simulink model "Control_test"  (R2014b)
settings: Solver=FixedStepDiscrete  StartTime=0.0  StopTime=Inf  FixedStep=0.001  RelTol=1e-3
PostLoadFcn:
  | , if any(exist('dsrtsu_mdlpostloadfcn', 'file') == [2, 3, 6]), try dsrtsu_mdlpostloadfcn('Execute', bdroot); catch fprintf('Error in PostLoadFcn (dsrtsu_mdlpostloadfcn) for model "%s":\n %s\n', bdroot, lasterr); end, end,
undefined symbols (not defined in the file or in its folder): dtLocal, slcm
libraries: rtican x163, simulink x14
(part 16 of 34)

== system Control_test/InputProcessing/RadarCanProcessing/MotionPower ==
  Bus Creator : BusCreator  Inputs=258
  Bus Creator1 : BusCreator  Inputs=64
  Bus Selector : BusSelector  OutputSignals=CAN_TX_TRACK_MOVING01,CAN_TX_TRACK_MOVING02,CAN_TX_TRACK_MOVING03,CAN_TX_TRACK_MOVING04,CAN_TX_TRACK_MOVING05,CAN_TX_TRACK_MOVING06,CAN_TX_TRACK_MOVING07,CAN_TX_TRACK_MOVING08,CAN_TX_TRACK_MOVING09,CAN_TX_TRACK_MOVING10,CAN_TX_TRACK_MOVING11,CAN_TX_TRACK_MOVING12,CAN_TX_TRACK_MOVING13,CAN_TX_TRACK_MOVING14,CAN_TX_TRACK_MOVING15,CAN_TX_TRACK_MOVING16,CAN_TX_TRACK_MOVING17,CAN_TX_TRACK_MOVING18,CAN_TX_TRACK_MOVING19,CAN_TX_TRACK_MOVING20,CAN_TX_TRACK_MOVING21,CAN_TX_TRACK_MOVING22,CAN_TX_TRACK_MOVING23,CAN_TX_TRACK_MOVING24,CAN_TX_TRACK_MOVING25,CAN_TX_TRACK_MOVING26,CAN_TX_TRACK_MOVING27,CAN_TX_TRACK_MOVING28,CAN_TX_TRACK_MOVING29,CAN_TX_TRACK_MOVING30,CAN_TX_TRACK_MOVING31,CAN_TX_TRACK_MOVING32,CAN_TX_TRACK_MOVING33,CAN_TX_TRACK_MOVING34,CAN_TX_TRACK_MOVING35,CAN_TX_TRACK_MOVING36,CAN_TX_TRACK_MOVING37,CAN_TX_TRACK_MOVING38,CAN_TX_TRACK_MOVING39,CAN_TX_TRACK_MOVING40,CAN_TX_TRACK_MOVING41,CAN_TX_TRACK_MOVING42,CAN_TX_TRACK_MOVING43,CAN_TX_TRACK_MOVING44,CAN_TX_TRACK_MOVING45,CAN_TX_TRACK_MOVING46,CAN_TX_TRACK_MOVING47,CAN_TX_TRACK_MOVING48,CAN_TX_TRACK_MOVING49,CAN_TX_TRACK_MOVING50,CAN_TX_TRACK_MOVING51,CAN_TX_TRACK_MOVING52,CAN_TX_TRACK_MOVING53,CAN_TX_TRACK_MOVING54,CAN_TX_TRACK_MOVING55,CAN_TX_TRACK_MOVING56,CAN_TX_TRACK_MOVING57,CAN_TX_TRACK_MOVING58,CAN_TX_TRACK_MOVING59,CAN_TX_TRACK_MOVING60,CAN_TX_TRACK_MOVING61,CAN_TX_TRACK_MOVING62,CAN_TX_TRACK_MOVING63,CAN_TX_TRACK_MOVING64
  ESR_TrackMotionPower : rtican/RTICAN Receive (RX)   Reserved1=[]  Reserved2=[]  Reserved3=[]  Reserved4=[]  SfcnMessage=[]  Msg_Struct=[]  BoardTypeNo=[]  BoardNo=[]  ChannelNo=[]  Parameters=[]  DialogFcn=[]  UnitName=[]  Revision=[]  UnitValues=[]  DSProperties=struct('RTI',struct('Version',uint32(5),'BlockType',struct('isSLSource',uint8(1),'isSLSink',uint8(1),'isHWSource',uint8(0),'isHWSink',uint8(0),'isSetup',uint8(0),'isInline',uint8(1),'isNonInline',uint8(0),'isInterrupt',uint8(0),'isChannelwise',uint8(0)),'IOBoardType','RTICAN','UnitType','MESSAGE','Identifier','RX','DialogType','MSVC','BlockSet','RTICAN','SlaveProcessor','CAN'))  RTIBlockInterface=struct('OutputPortsWidth',int32([1 1 1 1 1 1 1 1 1 1 1 1 1 1 1 1 1 1 1 1 1 1 1 1 1 1 1 1 1 1 1 1 1 1 1 1 1 1 1 1 1 1 1 1 1 1 1 1 1 1 1 1 1 1 1 1 1 1 1 1 1 1 1 1 1 1 1 1 1 1 1 1 1 1 1 1 1 1 1 1 1 1 1 1 1 1 1 1 1 1 1 1 1 1 1 1 1 1 1 1 1 1 1 1 1 1 1 1 1 1 1 1 1 1 1 1 1 1 1 1 1 1 1 1 1 1 1 1 1 1 1 1 1 1 1 1 1 1 1 1 1 1 1 1 1 1 1 1 1 1 1 1 1 1 1 1 1 1 1 1 1 1 1 1 1 1 1 1 1 1 1 1 1 1 1 1 1 1 1 1 1 1 1 1 1 1 1 1 1 1 1 1 1 1 1 1 1 1 1 1 1 1 1 1 1 1 1 1 1 1 1 1 1 1 1 1 1 1 1 1 1 1 1 1 1 1 1 1 1 1 1 1 1 1 1 1 1 1 1 1 1 1 1 1 1 1 1 1 1 1 1 1 1 1 1 1 1 1]),'OutputPortsActive',[1 1 1 1 1 1 1 1 1 1 1 1 1 1 1 1 1 1 1 1 1 1 1 1 1 1 1 1 1 1 1 1 1 1 1 1 1 1 1 1 1 1 1 1 1 1 1 1 1 1 1 1 1 1 1 1 1 1 1 1 1 1 1 1 1 1 1 1 1 1 1 1 1 1 1 1 1 1 1 1 1 1 1 1 1 1 1 1 1 1 1 1 1 1 1 1 1 1 1 1 1 1 1 1 1 1 1 1 1 1 1 1 1 1 1 1 1 1 1 1 1 1 1 1 1 1 1 1 1 1 1 1 1 1 1 1 1 1 1 1 1 1 1 1 1 1 1 1 1 1 1 1 1 1 1 1 1 1 1 1 1 1 1 1 1 1 1 1 1 1 1 1 1 1 1 1 1 1 1 1 1 1 1 1 1 1 1 1 1 1 1 1 1 1 1 1 1 1 1 1 1 1 1 1 1 1 1 1 1 1 1 1 1 1 1 1 1 1 1 1 1 1 1 1 1 1 1 1 1 1 1 1 1 1 1 1 1 1 1 1 1 1 1 1 1 1 1 1 1 1 1 1 1 1 1 1 1 1],'OutputPortsName',{{'CAN_TX_TRACK_POWER07','CAN_TX_TRACK_POWER14','CAN_TX_TRACK_POWER21','CAN_TX_TRACK_POWER28','CAN_TX_TRACK_POWER35','CAN_TX_TRACK_POWER42','CAN_TX_TRACK_POWER49','CAN_TX_TRACK_POWER56','CAN_TX_TRACK_POWER63','CAN_TX_TRACK_MOVING07','CAN_TX_TRACK_MOVING14','CAN_TX_TRACK_MOVING21','CAN_TX_TRACK_MOVING28','CAN_TX_TRACK_MOVING35','CAN_TX_TRACK_MOVING42','CAN_TX_TRACK_MOVING49','CAN_TX_TRACK_MOVING56','CAN_TX_TRACK_MOVING63','CAN_TX_TRACK_MOVABLE_SLOW07','CAN_TX_TRACK_MOVABLE_SLOW14','CAN_TX_TRACK_MOVABLE_SLOW21','CAN_TX_TRACK_MOVABLE_SLOW28','CAN_TX_TRACK_MOVABLE_SLOW35','CAN_TX_TRACK_MOVABLE_SLOW42','CAN_TX_TRACK_MOVABLE_SLOW49','CAN_TX_TRACK_MOVABLE_SLOW56','CAN_TX_TRACK_MOVABLE_SLOW63','CAN_TX_TRACK_MOVABLE_FAST07','CAN_TX_TRACK_MOVABLE_FAST14','CAN_TX_TRACK_MOVABLE_FAST21','CAN_TX_TRACK_MOVABLE_FAST28','CAN_TX_TRACK_MOVABLE_FAST35','CAN_TX_TRACK_MOVABLE_FAST42','CAN_TX_TRACK_MOVABLE_FAST49','CAN_TX_TRACK_MOVABLE_FAST56','CAN_TX_TRACK_MOVABLE_FAST63','CAN_TX_TRACK_POWER06','CAN_TX_TRACK_POWER13','CAN_TX_TRACK_POWER20','CAN_TX_TRACK_POWER27','CAN_TX_TRACK_POWER34','CAN_TX_TRACK_POWER41','CAN_TX_TRACK_POWER48','CAN_TX_TRACK_POWER55','CAN_TX_TRACK_POWER62','CAN_TX_TRACK_MOVING06','CAN_TX_TRACK_MOVING13','CAN_TX_TRACK_MOVING20','CAN_TX_TRACK_MOVING27','CAN_TX_TRACK_MOVING34','CAN_TX_TRACK_MOVING41','CAN_TX_TRACK_MOVING48','CAN_TX_TRACK_MOVING55','CAN_TX_TRACK_MOVING62','CAN_TX_TRACK_MOVABLE_SLOW06','CAN_TX_TRACK_MOVABLE_SLOW13','CAN_TX_TRACK_MOVABLE_SLOW20','CAN_TX_TRACK_MOVABLE_SLOW27','CAN_TX_TRACK_MOVABLE_SLOW34','CAN_TX_TRACK_MOVABLE_SLOW41','CAN_TX_TRACK_MOVABLE_SLOW48','CAN_TX_TRACK_MOVABLE_SLOW55','CAN_TX_TRACK_MOVABLE_SLOW62','CAN_TX_TRACK_MOVABLE_FAST06','CAN_TX_TRACK_MOVABLE_FAST13','CAN_TX_TRACK_MOVABLE_FAST20','CAN_TX_TRACK_MOVABLE_FAST27','CAN_TX_TRACK_MOVABLE_FAST34','CAN_TX_TRACK_MOVABLE_FAST41','CAN_TX_TRACK_MOVABLE_FAST48','CAN_TX_TRACK_MOVABLE_FAST55','CAN_TX_TRACK_MOVABLE_FAST62','CAN_TX_TRACK_POWER05','CAN_TX_TRACK_POWER12','CAN_TX_TRACK_POWER19','CAN_TX_TRACK_POWER26','CAN_TX_TRACK_POWER33','CAN_TX_TRACK_POWER40','CAN_TX_TRACK_POWER47','CAN_TX_TRACK_POWER54','CAN_TX_TRACK_POWER61','CAN_TX_TRACK_MOVING05','CAN_TX_TRACK_MOVING12','CAN_TX_TRACK_MOVING19','CAN_TX_TRACK_MOVING26','CAN_TX_TRACK_MOVING33','CAN_TX_TRACK_MOVING40','CAN_TX_TRACK_MOVING47','CAN_TX_TRACK_MOVING54','CAN_TX_TRACK_MOVING61','CAN_TX_TRACK_MOVABLE_SLOW05','CAN_TX_TRACK_MOVABLE_SLOW12','CAN_TX_TRACK_MOVABLE_SLOW19','CAN_TX_TRACK_MOVABLE_SLOW26','CAN_TX_TRACK_MOVABLE_SLOW33','CAN_TX_TRACK_MOVABLE_SLOW40','CAN_TX_TRACK_MOVABLE_SLOW47','CAN_TX_TRACK_MOVABLE_SLOW54','CAN_TX_TRACK_MOVABLE_SLOW61','CAN_TX_TRACK_MOVABLE_FAST05','CAN_TX_TRACK_MOVABLE_FAST12','CAN_TX_TRACK_MOVABLE_FAST19','CAN_TX_TRACK_MOVABLE_FAST26','CAN_TX_TRACK_MOVABLE_FAST33','CAN_TX_TRACK_MOVABLE_FAST40','CAN_TX_TRACK_MOVABLE_FAST47','CAN_TX_TRACK_MOVABLE_FAST54','CAN_TX_TRACK_MOVABLE_FAST61','CAN_TX_TRACK_POWER04','CAN_TX_TRACK_POWER11','CAN_TX_TRACK_POWER18','CAN_TX_TRACK_POWER25','CAN_TX_TRACK_POWER32','CAN_TX_TRACK_POWER39','CAN_TX_TRACK_POWER46','CAN_TX_TRACK_POWER53','CAN_TX_TRACK_POWER60','CAN_TX_TRACK_MOVING04','CAN_TX_TRACK_MOVING11','CAN_TX_TRACK_MOVING18','CAN_TX_TRACK_MOVING25','CAN_TX_TRACK_MOVING32','CAN_TX_TRACK_MOVING39','CAN_TX_TRACK_MOVING46','CAN_TX_TRACK_MOVING53','CAN_TX_TRACK_MOVING60','CAN_TX_TRACK_MOVABLE_SLOW04','CAN_TX_TRACK_MOVABLE_SLOW11','CAN_TX_TRACK_MOVABLE_SLOW18','CAN_TX_TRACK_MOVABLE_SLOW25','CAN_TX_TRACK_MOVABLE_SLOW32','CAN_TX_TRACK_MOVABLE_SLOW39','CAN_TX_TRACK_MOVABLE_SLOW46','CAN_TX_TRACK_MOVABLE_SLOW53','CAN_TX_TRACK_MOVABLE_SLOW60','CAN_TX_TRACK_MOVABLE_FAST04','CAN_TX_TRACK_MOVABLE_FAST11','CAN_TX_TRACK_MOVABLE_FAST18','CAN_TX_TRACK_MOVABLE_FAST25','CAN_TX_TRACK_MOVABLE_FAST32','CAN_TX_TRACK_MOVABLE_FAST39','CAN_TX_TRACK_MOVABLE_FAST46','CAN_TX_TRACK_MOVABLE_FAST53','CAN_TX_TRACK_MOVABLE_FAST60','CAN_TX_TRACK_POWER03','CAN_TX_TRACK_POWER10','CAN_TX_TRACK_POWER17','CAN_TX_TRACK_POWER24','CAN_TX_TRACK_POWER31','CAN_TX_TRACK_POWER38','CAN_TX_TRACK_POWER45','CAN_TX_TRACK_POWER52','CAN_TX_TRACK_POWER59','CAN_TX_TRACK_MOVING03','CAN_TX_TRACK_MOVING10','CAN_TX_TRACK_MOVING17','CAN_TX_TRACK_MOVING24','CAN_TX_TRACK_MOVING31','CAN_TX_TRACK_MOVING38','CAN_TX_TRACK_MOVING45','CAN_TX_TRACK_MOVING52','CAN_TX_TRACK_MOVING59','CAN_TX_TRACK_MOVABLE_SLOW03','CAN_TX_TRACK_MOVABLE_SLOW10','CAN_TX_TRACK_MOVABLE_SLOW17','CAN_TX_TRACK_MOVABLE_SLOW24','CAN_TX_TRACK_MOVABLE_SLOW31','CAN_TX_TRACK_MOVABLE_SLOW38','CAN_TX_TRACK_MOVABLE_SLOW45','CAN_TX_TRACK_MOVABLE_SLOW52','CAN_TX_TRACK_MOVABLE_SLOW59','CAN_TX_TRACK_MOVABLE_FAST03','CAN_TX_TRACK_MOVABLE_FAST10','CAN_TX_TRACK_MOVABLE_FAST17','CAN_TX_TRACK_MOVABLE_FAST24','CAN_TX_TRACK_MOVABLE_FAST31','CAN_TX_TRACK_MOVABLE_FAST38','CAN_TX_TRACK_MOVABLE_FAST45','CAN_TX_TRACK_MOVABLE_FAST52','CAN_TX_TRACK_MOVABLE_FAST59','CAN_TX_TRACK_POWER02','CAN_TX_TRACK_POWER09','CAN_TX_TRACK_POWER16','CAN_TX_TRACK_POWER23','CAN_TX_TRACK_POWER30','CAN_TX_TRACK_POWER37','CAN_TX_TRACK_POWER44','CAN_TX_TRACK_POWER51','CAN_TX_TRACK_POWER58','CAN_TX_TRACK_MOVING02','CAN_TX_TRACK_MOVING09','CAN_TX_TRACK_MOVING16','CAN_TX_TRACK_MOVING23','CAN_TX_TRACK_MOVING30','CAN_TX_TRACK_MOVING37','CAN_TX_TRACK_MOVING44','CAN_TX_TRACK_MOVING51','CAN_TX_TRACK_MOVING58','CAN_TX_TRACK_MOVABLE_SLOW02','CAN_TX_TRACK_MOVABLE_SLOW09','CAN_TX_TRACK_MOVABLE_SLOW16','CAN_TX_TRACK_MOVABLE_SLOW23','CAN_TX_TRACK_MOVABLE_SLOW30','CAN_TX_TRACK_MOVABLE_SLOW37','CAN_TX_TRACK_MOVABLE_SLOW44','CAN_TX_TRACK_MOVABLE_SLOW51','CAN_TX_TRACK_MOVABLE_SLOW58','CAN_TX_TRACK_MOVABLE_FAST02','CAN_TX_TRACK_MOVABLE_FAST09','CAN_TX_TRACK_MOVABLE_FAST16','CAN_TX_TRACK_MOVABLE_FAST23','CAN_TX_TRACK_MOVABLE_FAST30','CAN_TX_TRACK_MOVABLE_FAST37','CAN_TX_TRACK_MOVABLE_FAST44','CAN_TX_TRACK_MOVABLE_FAST51','CAN_TX_TRACK_MOVABLE_FAST58','CAN_TX_TRACK_POWER01','CAN_TX_TRACK_POWER08','CAN_TX_TRACK_POWER15','CAN_TX_TRACK_POWER22','CAN_TX_TRACK_POWER29','CAN_TX_TRACK_POWER36','CAN_TX_TRACK_POWER43','CAN_TX_TRACK_POWER50','CAN_TX_TRACK_POWER57','CAN_TX_TRACK_POWER64','CAN_TX_TRACK_MOVING01','CAN_TX_TRACK_MOVING08','CAN_TX_TRACK_MOVING15','CAN_TX_TRACK_MOVING22','CAN_TX_TRACK_MOVING29','CAN_TX_TRACK_MOVING36','CAN_TX_TRACK_MOVING43','CAN_TX_TRACK_MOVING50','CAN_TX_TRACK_MOVING57','CAN_TX_TRACK_MOVING64','CAN_TX_TRACK_MOVABLE_SLOW01','CAN_TX_TRACK_MOVABLE_SLOW08','CAN_TX_TRACK_MOVABLE_SLOW15','CAN_TX_TRACK_MOVABLE_SLOW22','CAN_TX_TRACK_MOVABLE_SLOW29','CAN_TX_TRACK_MOVABLE_SLOW36','CAN_TX_TRACK_MOVABLE_SLOW43','CAN_TX_TRACK_MOVABLE_SLOW50','CAN_TX_TRACK_MOVABLE_SLOW57','CAN_TX_TRACK_MOVABLE_SLOW64','CAN_TX_TRACK_MOVABLE_FAST01','CAN_TX_TRACK_MOVABLE_FAST08','CAN_TX_TRACK_MOVABLE_FAST15','CAN_TX_TRACK_MOVABLE_FAST22','CAN_TX_TRACK_MOVABLE_FAST29','CAN_TX_TRACK_MOVABLE_FAST36','CAN_TX_TRACK_MOVABLE_FAST43','CAN_TX_TRACK_MOVABLE_FAST50','CAN_TX_TRACK_MOVABLE_FAST57','CAN_TX_TRACK_MOVABLE_FAST64','CAN_TX_TRACK_CAN_ID_GROUP','CAN_TX_TRACK_ROLLING_COUNT_2'}},'OutputPortsDataType',{{'SS_DOUBLE','SS_DOUBLE','SS_DOUBLE','SS_DOUBLE','SS_DOUBLE','SS_DOUBLE','SS_DOUBLE','SS_DOUBLE','SS_DOUBLE','SS_DOUBLE','SS_DOUBLE','SS_DOUBLE','SS_DOUBLE','SS_DOUBLE','SS_DOUBLE','SS_DOUBLE','SS_DOUBLE','SS_DOUBLE','SS_DOUBLE','SS_DOUBLE','SS_DOUBLE','SS_DOUBLE','SS_DOUBLE','SS_DOUBLE','SS_DOUBLE','SS_DOUBLE','SS_DOUBLE','SS_DOUBLE','SS_DOUBLE','SS_DOUBLE','SS_DOUBLE','SS_DOUBLE','SS_DOUBLE','SS_DOUBLE','SS_DOUBLE','SS_DOUBLE','SS_DOUBLE','SS_DOUBLE','SS_DOUBLE','SS_DOUBLE','SS_DOUBLE','SS_DOUBLE','SS_DOUBLE','SS_DOUBLE','SS_DOUBLE','SS_DOUBLE','SS_DOUBLE','SS_DOUBLE','SS_DOUBLE','SS_DOUBLE','SS_DOUBLE','SS_DOUBLE','SS_DOUBLE','SS_DOUBLE','SS_DOUBLE','SS_DOUBLE','SS_DOUBLE','SS_DOUBLE','SS_DOUBLE','SS_DOUBLE','SS_DOUBLE','SS_DOUBLE','SS_DOUBLE','SS_DOUBLE','SS_DOUBLE','SS_DOUBLE','SS_DOUBLE','SS_DOUBLE','SS_DOUBLE','SS_DOUBLE','SS_DOUBLE','SS_DOUBLE','SS_DOUBLE','SS_DOUBLE','SS_DOUBLE','SS_DOUBLE','SS_DOUBLE','SS_DOUBLE','SS_DOUBLE','SS_DOUBLE','SS_DOUBLE','SS_DOUBLE','SS_DOUBLE','SS_DOUBLE','SS_DOUBLE','SS_DOUBLE','SS_DOUBLE','SS_DOUBLE','SS_DOUBLE','SS_DOUBLE','SS_DOUBLE','SS_DOUBLE','SS_DOUBLE','SS_DOUBLE','SS_DOUBLE','SS_DOUBLE','SS_DOUBLE','SS_DOUBLE','SS_DOUBLE','SS_DOUBLE','SS_DOUBLE','SS_DOUBLE','SS_DOUBLE','SS_DOUBLE','SS_DOUBLE','SS_DOUBLE','SS_DOUBLE','SS_DOUBLE','SS_DOUBLE','SS_DOUBLE','SS_DOUBLE','SS_DOUBLE','SS_DOUBLE','SS_DOUBLE','SS_DOUBLE','SS_DOUBLE','SS_DOUBLE','SS_DOUBLE','SS_DOUBLE','SS_DOUBLE','SS_DOUBLE','SS_DOUBLE','SS_DOUBLE','SS_DOUBLE','SS_DOUBLE','SS_DOUBLE','SS_DOUBLE','SS_DOUBLE','SS_DOUBLE','SS_DOUBLE','SS_DOUBLE','SS_DOUBLE','SS_DOUBLE','SS_DOUBLE','SS_DOUBLE','SS_DOUBLE','SS_DOUBLE','SS_DOUBLE','SS_DOUBLE','SS_DOUBLE','SS_DOUBLE','SS_DOUBLE','SS_DOUBLE','SS_DOUBLE','SS_DOUBLE','SS_DOUBLE','SS_DOUBLE','SS_DOUBLE','SS_DOUBLE','SS_DOUBLE','SS_DOUBLE','SS_DOUBLE','SS_DOUBLE','SS_DOUBLE','SS_DOUBLE','SS_DOUBLE','SS_DOUBLE','SS_DOUBLE','SS_DOUBLE','SS_DOUBLE','SS_DOUBLE','SS_DOUBLE','SS_DOUBLE','SS_DOUBLE','SS_DOUBLE','SS_DOUBLE','SS_DOUBLE','SS_DOUBLE','SS_DOUBLE','SS_DOUBLE','SS_DOUBLE','SS_DOUBLE','SS_DOUBLE','SS_DOUBLE','SS_DOUBLE','SS_DOUBLE','SS_DOUBLE','SS_DOUBLE','SS_DOUBLE','SS_DOUBLE','SS_DOUBLE','SS_DOUBLE','SS_DOUBLE','SS_DOUBLE','SS_DOUBLE','SS_DOUBLE','SS_DOUBLE','SS_DOUBLE','SS_DOUBLE','SS_DOUBLE','SS_DOUBLE','SS_DOUBLE','SS_DOUBLE','SS_DOUBLE','SS_DOUBLE','SS_DOUBLE','SS_DOUBLE','SS_DOUBLE','SS_DOUBLE','SS_DOUBLE','SS_DOUBLE','SS_DOUBLE','SS_DOUBLE','SS_DOUBLE','SS_DOUBLE','SS_DOUBLE','SS_DOUBLE','SS_DOUBLE','SS_DOUBLE','SS_DOUBLE','SS_DOUBLE','SS_DOUBLE','SS_DOUBLE','SS_DOUBLE','SS_DOUBLE','SS_DOUBLE','SS_DOUBLE','SS_DOUBLE','SS_DOUBLE','SS_DOUBLE','SS_DOUBLE','SS_DOUBLE','SS_DOUBLE','SS_DOUBLE','SS_DOUBLE','SS_DOUBLE','SS_DOUBLE','SS_DOUBLE','SS_DOUBLE','SS_DOUBLE','SS_DOUBLE','SS_DOUBLE','SS_DOUBLE','SS_DOUBLE','SS_DOUBLE','SS_DOUBLE','SS_DOUBLE','SS_DOUBLE','SS_DOUBLE','SS_DOUBLE','SS_DOUBLE','SS_DOUBLE','SS_DOUBLE','SS_DOUBLE','SS_DOUBLE','SS_DOUBLE','SS_DOUBLE','SS_DOUBLE','SS_DOUBLE','SS_DOUBLE','SS_DOUBLE','SS_DOUBLE','SS_DOUBLE','SS_DOUBLE','SS_DOUBLE','SS_DOUBLE','SS_DOUBLE','SS_DOUBLE'}},'OutputPortsLabel',{{'CAN_TX_TRACK_POWER07','CAN_TX_TRACK_POWER14','CAN_TX_TRACK_POWER21','CAN_TX_TRACK_POWER28','CAN_TX_TRACK_POWER35','CAN_TX_TRACK_POWER42','CAN_TX_TRACK_POWER49','CAN_TX_TRACK_POWER56','CAN_TX_TRACK_POWER63','CAN_TX_TRACK_MOVING07','CAN_TX_TRACK_MOVING14','CAN_TX_TRACK_MOVING21','CAN_TX_TRACK_MOVING28','CAN_TX_TRACK_MOVING35','CAN_TX_TRACK_MOVING42','CAN_TX_TRACK_MOVING49','CAN_TX_TRACK_MOVING56','CAN_TX_TRACK_MOVING63','CAN_TX_TRACK_MOVABLE_SLOW07','CAN_TX_TRACK_MOVABLE_SLOW14','CAN_TX_TRACK_MOVABLE_SLOW21','CAN_TX_TRACK_MOVABLE_SLOW28','CAN_TX_TRACK_MOVABLE_SLOW35','CAN_TX_TRACK_MOVABLE_SLOW42','CAN_TX_TRACK_MOVABLE_SLOW49','CAN_TX_TRACK_MOVABLE_SLOW56','CAN_TX_TRACK_MOVABLE_SLOW63','CAN_TX_TRACK_MOVABLE_FAST07','CAN_TX_TRACK_MOVABLE_FAST14','CAN_TX_TRACK_MOVABLE_FAST21','CAN_TX_TRACK_MOVABLE_FAST28','CAN_TX_TRACK_MOVABLE_FAST35','CAN_TX_TRACK_MOVABLE_FAST42','CAN_TX_TRACK_MOVABLE_FAST49','CAN_TX_TRACK_MOVABLE_FAST56','CAN_TX_TRACK_MOVABLE_FAST63','CAN_TX_TRACK_POWER06','CAN_TX_TRACK_POWER13','CAN_TX_TRACK_POWER20','CAN_TX_TRACK_POWER27','CAN_TX_TRACK_POWER34','CAN_TX_TRACK_POWER41','CAN_TX_TRACK_POWER48','CAN_TX_TRACK_POWER55','CAN_TX_TRACK_POWER62','CAN_TX_TRACK_MOVING06','CAN_TX_TRACK_MOVING13','CAN_TX_TRACK_MOVING20','CAN_TX_TRACK_MOVING27','CAN_TX_TRACK_MOVING34','CAN_TX_TRACK_MOVING41','CAN_TX_TRACK_MOVING48','CAN_TX_TRACK_MOVING55','CAN_TX_TRACK_MOVING62','CAN_TX_TRACK_MOVABLE_SLOW06','CAN_TX_TRACK_MOVABLE_SLOW13','CAN_TX_TRACK_MOVABLE_SLOW20','CAN_TX_TRACK_MOVABLE_SLOW27','CAN_TX_TRACK_MOVABLE_SLOW34','CAN_TX_TRACK_MOVABLE_SLOW41','CAN_TX_TRACK_MOVABLE_SLOW48','CAN_TX_TRACK_MOVABLE_SLOW55','CAN_TX_TRACK_MOVABLE_SLOW62','CAN_TX_TRACK_MOVABLE_FAST06','CAN_TX_TRACK_MOVABLE_FAST13','CAN_TX_TRACK_MOVABLE_FAST20','CAN_TX_TRACK_MOVABLE_FAST27','CAN_TX_TRACK_MOVABLE_FAST34','CAN_TX_TRACK_MOVABLE_FAST41','CAN_TX_TRACK_MOVABLE_FAST48','CAN_TX_TRACK_MOVABLE_FAST55','CAN_TX_TRACK_MOVABLE_FAST62','CAN_TX_TRACK_POWER05','CAN_TX_TRACK_POWER12','CAN_TX_TRACK_POWER19','CAN_TX_TRACK_POWER26','CAN_TX_TRACK_POWER33','CAN_TX_TRACK_POWER40','CAN_TX_TRACK_POWER47','CAN_TX_TRACK_POWER54','CAN_TX_TRACK_POWER61','CAN_TX_TRACK_MOVING05','CAN_TX_TRACK_MOVING12','CAN_TX_TRACK_MOVING19','CAN_TX_TRACK_MOVING26','CAN_TX_TRACK_MOVING33','CAN_TX_TRACK_MOVING40','CAN_TX_TRACK_MOVING47','CAN_TX_TRACK_MOVING54','CAN_TX_TRACK_MOVING61','CAN_TX_TRACK_MOVABLE_SLOW05','CAN_TX_TRACK_MOVABLE_SLOW12','CAN_TX_TRACK_MOVABLE_SLOW19','CAN_TX_TRACK_MOVABLE_SLOW26','CAN_TX_TRACK_MOVABLE_SLOW33','CAN_TX_TRACK_MOVABLE_SLOW40','CAN_TX_TRACK_MOVABLE_SLOW47','CAN_TX_TRACK_MOVABLE_SLOW54','CAN_TX_TRACK_MOVABLE_SLOW61','CAN_TX_TRACK_MOVABLE_FAST05','CAN_TX_TRACK_MOVABLE_FAST12','CAN_TX_TRACK_MOVABLE_FAST19','CAN_TX_TRACK_MOVABLE_FAST26','CAN_TX_TRACK_MOVABLE_FAST33','CAN_TX_TRACK_MOVABLE_FAST40','CAN_TX_TRACK_MOVABLE_FAST47','CAN_TX_TRACK_MOVABLE_FAST54','CAN_TX_TRACK_MOVABLE_FAST61','CAN_TX_TRACK_POWER04','CAN_TX_TRACK_POWER11','CAN_TX_TRACK_POWER18','CAN_TX_TRACK_POWER25','CAN_TX_TRACK_POWER32','CAN_TX_TRACK_POWER39','CAN_TX_TRACK_POWER46','CAN_TX_TRACK_POWER53','CAN_TX_TRACK_POWER60','CAN_TX_TRACK_MOVING04','CAN_TX_TRACK_MOVING11','CAN_TX_TRACK_MOVING18','CAN_TX_TRACK_MOVING25','CAN_TX_TRACK_MOVING32','CAN_TX_TRACK_MOVING39','CAN_TX_TRACK_MOVING46','CAN_TX_TRACK_MOVING53','CAN_TX_TRACK_MOVING60','CAN_TX_TRACK_MOVABLE_SLOW04','CAN_TX_TRACK_MOVABLE_SLOW11','CAN_TX_TRACK_MOVABLE_SLOW18','CAN_TX_TRACK_MOVABLE_SLOW25','CAN_TX_TRACK_MOVABLE_SLOW32','CAN_TX_TRACK_MOVABLE_SLOW39','CAN_TX_TRACK_MOVABLE_SLOW46','CAN_TX_TRACK_MOVABLE_SLOW53','CAN_TX_TRACK_MOVABLE_SLOW60','CAN_TX_TRACK_MOVABLE_FAST04','CAN_TX_TRACK_MOVABLE_FAST11','CAN_TX_TRACK_MOVABLE_FAST18','CAN_TX_TRACK_MOVABLE_FAST25','CAN_TX_TRACK_MOVABLE_FAST32','CAN_TX_TRACK_MOVABLE_FAST39','CAN_TX_TRACK_MOVABLE_FAST46','CAN_TX_TRACK_MOVABLE_FAST53','CAN_TX_TRACK_MOVABLE_FAST60','CAN_TX_TRACK_POWER03','CAN_TX_TRACK_POWER10','CAN_TX_TRACK_POWER17','CAN_TX_TRACK_POWER24','CAN_TX_TRACK_POWER31','CAN_TX_TRACK_POWER38','CAN_TX_TRACK_POWER45','CAN_TX_TRACK_POWER52','CAN_TX_TRACK_POWER59','CAN_TX_TRACK_MOVING03','CAN_TX_TRACK_MOVING10','CAN_TX_TRACK_MOVING17','CAN_TX_TRACK_MOVING24','CAN_TX_TRACK_MOVING31','CAN_TX_TRACK_MOVING38','CAN_TX_TRACK_MOVING45','CAN_TX_TRACK_MOVING52','CAN_TX_TRACK_MOVING59','CAN_TX_TRACK_MOVABLE_SLOW03','CAN_TX_TRACK_MOVABLE_SLOW10','CAN_TX_TRACK_MOVABLE_SLOW17','CAN_TX_TRACK_MOVABLE_SLOW24','CAN_TX_TRACK_MOVABLE_SLOW31','CAN_TX_TRACK_MOVABLE_SLOW38','CAN_TX_TRACK_MOVABLE_SLOW45','CAN_TX_TRACK_MOVABLE_SLOW52','CAN_TX_TRACK_MOVABLE_SLOW59','CAN_TX_TRACK_MOVABLE_FAST03','CAN_TX_TRACK_MOVABLE_FAST10','CAN_TX_TRACK_MOVABLE_FAST17','CAN_TX_TRACK_MOVABLE_FAST24','CAN_TX_TRACK_MOVABLE_FAST31','CAN_TX_TRACK_MOVABLE_FAST38','CAN_TX_TRACK_MOVABLE_FAST45','CAN_TX_TRACK_MOVABLE_FAST52','CAN_TX_TRACK_MOVABLE_FAST59','CAN_TX_TRACK_POWER02','CAN_TX_TRACK_POWER09','CAN_TX_TRACK_POWER16','CAN_TX_TRACK_POWER23','CAN_TX_TRACK_POWER30','CAN_TX_TRACK_POWER37','CAN_TX_TRACK_POWER44','CAN_TX_TRACK_POWER51','CAN_TX_TRACK_POWER58','CAN_TX_TRACK_MOVING02','CAN_TX_TRACK_MOVING09','CAN_TX_TRACK_MOVING16','CAN_TX_TRACK_MOVING23','CAN_TX_TRACK_MOVING30','CAN_TX_TRACK_MOVING37','CAN_TX_TRACK_MOVING44','CAN_TX_TRACK_MOVING51','CAN_TX_TRACK_MOVING58','CAN_TX_TRACK_MOVABLE_SLOW02','CAN_TX_TRACK_MOVABLE_SLOW09','CAN_TX_TRACK_MOVABLE_SLOW16','CAN_TX_TRACK_MOVABLE_SLOW23','CAN_TX_TRACK_MOVABLE_SLOW30','CAN_TX_TRACK_MOVABLE_SLOW37','CAN_TX_TRACK_MOVABLE_SLOW44','CAN_TX_TRACK_MOVABLE_SLOW51','CAN_TX_TRACK_MOVABLE_SLOW58','CAN_TX_TRACK_MOVABLE_FAST02','CAN_TX_TRACK_MOVABLE_FAST09','CAN_TX_TRACK_MOVABLE_FAST16','CAN_TX_TRACK_MOVABLE_FAST23','CAN_TX_TRACK_MOVABLE_FAST30','CAN_TX_TRACK_MOVABLE_FAST37','CAN_TX_TRACK_MOVABLE_FAST44','CAN_TX_TRACK_MOVABLE_FAST51','CAN_TX_TRACK_MOVABLE_FAST58','CAN_TX_TRACK_POWER01','CAN_TX_TRACK_POWER08','CAN_TX_TRACK_POWER15','CAN_TX_TRACK_POWER22','CAN_TX_TRACK_POWER29','CAN_TX_TRACK_POWER36','CAN_TX_TRACK_POWER43','CAN_TX_TRACK_POWER50','CAN_TX_TRACK_POWER57','CAN_TX_TRACK_POWER64','CAN_TX_TRACK_MOVING01','CAN_TX_TRACK_MOVING08','CAN_TX_TRACK_MOVING15','CAN_TX_TRACK_MOVING22','CAN_TX_TRACK_MOVING29','CAN_TX_TRACK_MOVING36','CAN_TX_TRACK_MOVING43','CAN_TX_TRACK_MOVING50','CAN_TX_TRACK_MOVING57','CAN_TX_TRACK_MOVING64','CAN_TX_TRACK_MOVABLE_SLOW01','CAN_TX_TRACK_MOVABLE_SLOW08','CAN_TX_TRACK_MOVABLE_SLOW15','CAN_TX_TRACK_MOVABLE_SLOW22','CAN_TX_TRACK_MOVABLE_SLOW29','CAN_TX_TRACK_MOVABLE_SLOW36','CAN_TX_TRACK_MOVABLE_SLOW43','CAN_TX_TRACK_MOVABLE_SLOW50','CAN_TX_TRACK_MOVABLE_SLOW57','CAN_TX_TRACK_MOVABLE_SLOW64','CAN_TX_TRACK_MOVABLE_FAST01','CAN_TX_TRACK_MOVABLE_FAST08','CAN_TX_TRACK_MOVABLE_FAST15','CAN_TX_TRACK_MOVABLE_FAST22','CAN_TX_TRACK_MOVABLE_FAST29','CAN_TX_TRACK_MOVABLE_FAST36','CAN_TX_TRACK_MOVABLE_FAST43','CAN_TX_TRACK_MOVABLE_FAST50','CAN_TX_TRACK_MOVABLE_FAST57','CAN_TX_TRACK_MOVABLE_FAST64','CAN_TX_TRACK_CAN_ID_GROUP','CAN_TX_TRACK_ROLLING_COUNT_2'}},'OutputPortsLabelMode','ON','InputPortsWidth',int32(0),'InputPortsActive',0,'DialogFcn','rtican_message_interface_gui','BlockDisplay',{{'','center'}},'IconTransparency','on','ParameterTunableNames',{{}},'InitLevel',3,'BlockName',struct('Token',{{'ESR_TrackMotionPower'}}),'SampleTime',{{0.01}},'TriggerPort',{{'none'}},'EnablePort',{{'none'}})  RTIBlockParameters=struct('BoardTypeNo',{{1,'OFF',[]}},'BoardNo',{{2,'ON',[1 16]}},'ChannelNo',{{2,'ON',[1 2]}},'Parameters',{{struct('DataFileSupport',struct('DataFileSelectedMaster',1,'DataFileSelectedLocal',1,'DataFileName','c:\users\mpc_car\documents\github\mpc-car\controller\dbcfiles\esr_dv3_64tgt.dbc|','DataFileDate',['26-Aug-2014 13:16:21'],'SelectedFile','..\..\dbcfiles\esr_dv3_64tgt.dbc','InterfaceFcn','rtican_dbc_file_parser'),'Options',struct('StatusSelected',0,'TimeSelected',0,'DeltaTimeSelected',0,'BytePortSelected',0,'MessageLengthSelected',0,'TriggerPort',struct('Selected',0,'TriggerType',0),'UserCoding',struct('Selected',0,'InterfaceFile','UserDecodingFile','FcnName','UserDecodeFcn','InportSelected',0,'InportWidth',1,'OutportSelected',0,'OutportWidth',1),'EnablePortSelected',0,'SignalOnPortnameSelected',1,'UseRXService',0),'Message',struct('MsgOnBlocknameSelected',1,'MsgName','ESR_TrackMotionPower','MsgIdFormat',0,'MsgId',1344,'MsgLength',8,'NumSignals',258,'SampleTime',0.01,'Signal',struct('SgnName',{'CAN_TX_TRACK_POWER07','CAN_TX_TRACK_POWER14','CAN_TX_TRACK_POWER21','CAN_TX_TRACK_POWER28','CAN_TX_TRACK_POWER35','CAN_TX_TRACK_POWER42','CAN_TX_TRACK_POWER49','CAN_TX_TRACK_POWER56','CAN_TX_TRACK_POWER63','CAN_TX_TRACK_MOVING07','CAN_TX_TRACK_MOVING14','CAN_TX_TRACK_MOVING21','CAN_TX_TRACK_MOVING28','CAN_TX_TRACK_MOVING35','CAN_TX_TRACK_MOVING42','CAN_TX_TRACK_MOVING49','CAN_TX_TRACK_MOVING56','CAN_TX_TRACK_MOVING63','CAN_TX_TRACK_MOVABLE_SLOW07','CAN_TX_TRACK_MOVABLE_SLOW14','CAN_TX_TRACK_MOVABLE_SLOW21','CAN_TX_TRACK_MOVABLE_SLOW28','CAN_TX_TRACK_MOVABLE_SLOW35','CAN_TX_TRACK_MOVABLE_SLOW42','CAN_TX_TRACK_MOVABLE_SLOW49','CAN_TX_TRACK_MOVABLE_SLOW56','CAN_TX_TRACK_MOVABLE_SLOW63','CAN_TX_TRACK_MOVABLE_FAST07','CAN_TX_TRACK_MOVABLE_FAST14','CAN_TX_TRACK_MOVABLE_FAST21','CAN_TX_TRACK_MOVABLE_FAST28','CAN_TX_TRACK_MOVABLE_FAST35','CAN_TX_TRACK_MOVABLE_FAST42','CAN_TX_TRACK_MOVABLE_FAST49','CAN_TX_TRACK_MOVABLE_FAST56','CAN_TX_TRACK_MOVABLE_FAST63','CAN_TX_TRACK_POWER06','CAN_TX_TRACK_POWER13','CAN_TX_TRACK_POWER20','CAN_TX_TRACK_POWER27','CAN_TX_TRACK_POWER34','CAN_TX_TRACK_POWER41','CAN_TX_TRACK_POWER48','CAN_TX_TRACK_POWER55','CAN_TX_TRACK_POWER62','CAN_TX_TRACK_MOVING06','CAN_TX_TRACK_MOVING13','CAN_TX_TRACK_MOVING20','CAN_TX_TRACK_MOVING27','CAN_TX_TRACK_MOVING34','CAN_TX_TRACK_MOVING41','CAN_TX_TRACK_MOVING48','CAN_TX_TRACK_MOVING55','CAN_TX_TRACK_MOVING62','CAN_TX_TRACK_MOVABLE_SLOW06','CAN_TX_TRACK_MOVABLE_SLOW13','CAN_TX_TRACK_MOVABLE_SLOW20','CAN_TX_TRACK_MOVABLE_SLOW27','CAN_TX_TRACK_MOVABLE_SLOW34','CAN_TX_TRACK_MOVABLE_SLOW41','CAN_TX_TRACK_MOVABLE_SLOW48','CAN_TX_TRACK_MOVABLE_SLOW55','CAN_TX_TRACK_MOVABLE_SLOW62','CAN_TX_TRACK_MOVABLE_FAST06','CAN_TX_TRACK_MOVABLE_FAST13','CAN_TX_TRACK_MOVABLE_FAST20','CAN_TX_TRACK_MOVABLE_FAST27','CAN_TX_TRACK_MOVABLE_FAST34','CAN_TX_TRACK_MOVABLE_FAST41','CAN_TX_TRACK_MOVABLE_FAST48','CAN_TX_TRACK_MOVABLE_FAST55','CAN_TX_TRACK_MOVABLE_FAST62','CAN_TX_TRACK_POWER05','CAN_TX_TRACK_POWER12','CAN_TX_TRACK_POWER19','CAN_TX_TRACK_POWER26','CAN_TX_TRACK_POWER33','CAN_TX_TRACK_POWER40','CAN_TX_TRACK_POWER47','CAN_TX_TRACK_POWER54','CAN_TX_TRACK_POWER61','CAN_TX_TRACK_MOVING05','CAN_TX_TRACK_MOVING12','CAN_TX_TRACK_MOVING19','CAN_TX_TRACK_MOVING26','CAN_TX_TRACK_MOVING33','CAN_TX_TRACK_MOVING40','CAN_TX_TRACK_MOVING47','CAN_TX_TRACK_MOVING54','CAN_TX_TRACK_MOVING61','CAN_TX_TRACK_MOVABLE_SLOW05','CAN_TX_TRACK_MOVABLE_SLOW12','CAN_TX_TRACK_MOVABLE_SLOW19','CAN_TX_TRACK_MOVABLE_SLOW26','CAN_TX_TRACK_MOVABLE_SLOW33','CAN_TX_TRACK_MOVABLE_SLOW40','CAN_TX_TRACK_MOVABLE_SLOW47','CAN_TX_TRACK_MOVABLE_SLOW54','CAN_TX_TRACK_MOVABLE_SLOW61','CAN_TX_TRACK_MOVABLE_FAST05','CAN_TX_TRACK_MOVABLE_FAST12','CAN_TX_TRACK_MOVABLE_FAST19','CAN_TX_TRACK_MOVABLE_FAST26','CAN_TX_TRACK_MOVABLE_FAST33','CAN_TX_TRACK_MOVABLE_FAST40','CAN_TX_TRACK_MOVABLE_FAST47','CAN_TX_TRACK_MOVABLE_FAST54','CAN_TX_TRACK_MOVABLE_FAST61','CAN_TX_TRACK_POWER04','CAN_TX_TRACK_POWER11','CAN_TX_TRACK_POWER18','CAN_TX_TRACK_POWER25','CAN_TX_TRACK_POWER32','CAN_TX_TRACK_POWER39','CAN_TX_TRACK_POWER46','CAN_TX_TRACK_POWER53','CAN_TX_TRACK_POWER60','CAN_TX_TRACK_MOVING04','CAN_TX_TRACK_MOVING11','CAN_TX_TRACK_MOVING18','CAN_TX_TRACK_MOVING25','CAN_TX_TRACK_MOVING32','CAN_TX_TRACK_MOVING39','CAN_TX_TRACK_MOVING46','CAN_TX_TRACK_MOVING53','CAN_TX_TRACK_MOVING60','CAN_TX_TRACK_MOVABLE_SLOW04','CAN_TX_TRACK_MOVABLE_SLOW11','CAN_TX_TRACK_MOVABLE_SLOW18','CAN_TX_TRACK_MOVABLE_SLOW25','CAN_TX_TRACK_MOVABLE_SLOW32','CAN_TX_TRACK_MOVABLE_SLOW39','CAN_TX_TRACK_MOVABLE_SLOW46','CAN_TX_TRACK_MOVABLE_SLOW53','CAN_TX_TRACK_MOVABLE_SLOW60','CAN_TX_TRACK_MOVABLE_FAST04','CAN_TX_TRACK_MOVABLE_FAST11','CAN_TX_TRACK_MOVABLE_FAST18','CAN_TX_TRACK_MOVABLE_FAST25','CAN_TX_TRACK_MOVABLE_FAST32','CAN_TX_TRACK_MOVABLE_FAST39','CAN_TX_TRACK_MOVABLE_FAST46','CAN_TX_TRACK_MOVABLE_FAST53','CAN_TX_TRACK_MOVABLE_FAST60','CAN_TX_TRACK_POWER03','CAN_TX_TRACK_POWER10','CAN_TX_TRACK_POWER17','CAN_TX_TRACK_POWER24','CAN_TX_TRACK_POWER31','CAN_TX_TRACK_POWER38','CAN_TX_TRACK_POWER45','CAN_TX_TRACK_POWER52','CAN_TX_TRACK_POWER59','CAN_TX_TRACK_MOVING03','CAN_TX_TRACK_MOVING10','CAN_TX_TRACK_MOVING17','CAN_TX_TRACK_MOVING24','CAN_TX_TRACK_MOVING31','CAN_TX_TRACK_MOVING38','CAN_TX_TRACK_MOVING45','CAN_TX_TRACK_MOVING52','CAN_TX_TRACK_MOVING59','CAN_TX_TRACK_MOVABLE_SLOW03','CAN_TX_TRACK_MOVABLE_SLOW10','CAN_TX_TRACK_MOVABLE_SLOW17','CAN_TX_TRACK_MOVABLE_SLOW24','CAN_TX_TRACK_MOVABLE_SLOW31','CAN_TX_TRACK_MOVABLE_SLOW38','CAN_TX_TRACK_MOVABLE_SLOW45','CAN_TX_TRACK_MOVABLE_SLOW52','CAN_TX_TRACK_MOVABLE_SLOW59','CAN_TX_TRACK_MOVABLE_FAST03','CAN_TX_TRACK_MOVABLE_FAST10','CAN_TX_TRACK_MOVABLE_FAST17','CAN_TX_TRACK_MOVABLE_FAST24','CAN_TX_TRACK_MOVABLE_FAST31','CAN_TX_TRACK_MOVABLE_FAST38','CAN_TX_TRACK_MOVABLE_FAST45','CAN_TX_TRACK_MOVABLE_FAST52','CAN_TX_TRACK_MOVABLE_FAST59','CAN_TX_TRACK_POWER02','CAN_TX_TRACK_POWER09','CAN_TX_TRACK_POWER16','CAN_TX_TRACK_POWER23','CAN_TX_TRACK_POWER30','CAN_TX_TRACK_POWER37','CAN_TX_TRACK_POWER44','CAN_TX_TRACK_POWER51','CAN_TX_TRACK_POWER58','CAN_TX_TRACK_MOVING02','CAN_TX_TRACK_MOVING09','CAN_TX_TRACK_MOVING16','CAN_TX_TRACK_MOVING23','CAN_TX_TRACK_MOVING30','CAN_TX_TRACK_MOVING37','CAN_TX_TRACK_MOVING44','CAN_TX_TRACK_MOVING51','CAN_TX_TRACK_MOVING58','CAN_TX_TRACK_MOVABLE_SLOW02','CAN_TX_TRACK_MOVABLE_SLOW09','CAN_TX_TRACK_MOVABLE_SLOW16','CAN_TX_TRACK_MOVABLE_SLOW23','CAN_TX_TRACK_MOVABLE_SLOW30','CAN_TX_TRACK_MOVABLE_SLOW37','CAN_TX_TRACK_MOVABLE_SLOW44','CAN_TX_TRACK_MOVABLE_SLOW51','CAN_TX_TRACK_MOVABLE_SLOW58','CAN_TX_TRACK_MOVABLE_FAST02','CAN_TX_TRACK_MOVABLE_FAST09','CAN_TX_TRACK_MOVABLE_FAST16','CAN_TX_TRACK_MOVABLE_FAST23','CAN_TX_TRACK_MOVABLE_FAST30','CAN_TX_TRACK_MOVABLE_FAST37','CAN_TX_TRACK_MOVABLE_FAST44','CAN_TX_TRACK_MOVABLE_FAST51','CAN_TX_TRACK_MOVABLE_FAST58','CAN_TX_TRACK_POWER01','CAN_TX_TRACK_POWER08','CAN_TX_TRACK_POWER15','CAN_TX_TRACK_POWER22','CAN_TX_TRACK_POWER29','CAN_TX_TRACK_POWER36','CAN_TX_TRACK_POWER43','CAN_TX_TRACK_POWER50','CAN_TX_TRACK_POWER57','CAN_TX_TRACK_POWER64','CAN_TX_TRACK_MOVING01','CAN_TX_TRACK_MOVING08','CAN_TX_TRACK_MOVING15','CAN_TX_TRACK_MOVING22','CAN_TX_TRACK_MOVING29','CAN_TX_TRACK_MOVING36','CAN_TX_TRACK_MOVING43','CAN_TX_TRACK_MOVING50','CAN_TX_TRACK_MOVING57','CAN_TX_TRACK_MOVING64','CAN_TX_TRACK_MOVABLE_SLOW01','CAN_TX_TRACK_MOVABLE_SLOW08','CAN_TX_TRACK_MOVABLE_SLOW15','CAN_TX_TRACK_MOVABLE_SLOW22','CAN_TX_TRACK_MOVABLE_SLOW29','CAN_TX_TRACK_MOVABLE_SLOW36','CAN_TX_TRACK_MOVABLE_SLOW43','CAN_TX_TRACK_MOVABLE_SLOW50','CAN_TX_TRACK_MOVABLE_SLOW57','CAN_TX_TRACK_MOVABLE_SLOW64','CAN_TX_TRACK_MOVABLE_FAST01','CAN_TX_TRACK_MOVABLE_FAST08','CAN_TX_TRACK_MOVABLE_FAST15','CAN_TX_TRACK_MOVABLE_FAST22','CAN_TX_TRACK_MOVABLE_FAST29','CAN_TX_TRACK_MOVABLE_FAST36','CAN_TX_TRACK_MOVABLE_FAST43','CAN_TX_TRACK_MOVABLE_FAST50','CAN_TX_TRACK_MOVABLE_FAST57','CAN_TX_TRACK_MOVABLE_FAST64','CAN_TX_TRACK_CAN_ID_GROUP','CAN_TX_TRACK_ROLLING_COUNT_2'},'SgnStartBit',{0,0,0,0,0,0,0,0,0,5,5,5,5,5,5,5,5,5,6,6,6,6,6,6,6,6,6,7,7,7,7,7,7,7,7,7,8,8,8,8,8,8,8,8,8,13,13,13,13,13,13,13,13,13,14,14,14,14,14,14,14,14,14,15,15,15,15,15,15,15,15,15,16,16,16,16,16,16,16,16,16,21,21,21,21,21,21,21,21,21,22,22,22,22,22,22,22,22,22,23,23,23,23,23,23,23,23,23,24,24,24,24,24,24,24,24,24,29,29,29,29,29,29,29,29,29,30,30,30,30,30,30,30,30,30,31,31,31,31,31,31,31,31,31,32,32,32,32,32,32,32,32,32,37,37,37,37,37,37,37,37,37,38,38,38,38,38,38,38,38,38,39,39,39,39,39,39,39,39,39,40,40,40,40,40,40,40,40,40,45,45,45,45,45,45,45,45,45,46,46,46,46,46,46,46,46,46,47,47,47,47,47,47,47,47,47,48,48,48,48,48,48,48,48,48,48,53,53,53,53,53,53,53,53,53,53,54,54,54,54,54,54,54,54,54,54,55,55,55,55,55,55,55,55,55,55,56,60},'SgnLength',{5,5,5,5,5,5,5,5,5,1,1,1,1,1,1,1,1,1,1,1,1,1,1,1,1,1,1,1,1,1,1,1,1,1,1,1,5,5,5,5,5,5,5,5,5,1,1,1,1,1,1,1,1,1,1,1,1,1,1,1,1,1,1,1,1,1,1,1,1,1,1,1,5,5,5,5,5,5,5,5,5,1,1,1,1,1,1,1,1,1,1,1,1,1,1,1,1,1,1,1,1,1,1,1,1,1,1,1,5,5,5,5,5,5,5,5,5,1,1,1,1,1,1,1,1,1,1,1,1,1,1,1,1,1,1,1,1,1,1,1,1,1,1,1,5,5,5,5,5,5,5,5,5,1,1,1,1,1,1,1,1,1,1,1,1,1,1,1,1,1,1,1,1,1,1,1,1,1,1,1,5,5,5,5,5,5,5,5,5,1,1,1,1,1,1,1,1,1,1,1,1,1,1,1,1,1,1,1,1,1,1,1,1,1,1,1,5,5,5,5,5,5,5,5,5,5,1,1,1,1,1,1,1,1,1,1,1,1,1,1,1,1,1,1,1,1,1,1,1,1,1,1,1,1,1,1,4,1},'ByteLayout',{2,2,2,2,2,2,2,2,2,2,2,2,2,2,2,2,2,2,2,2,2,2,2,2,2,2,2,2,2,2,2,2,2,2,2,2,2,2,2,2,2,2,2,2,2,2,2,2,2,2,2,2,2,2,2,2,2,2,2,2,2,2,2,2,2,2,2,2,2,2,2,2,2,2,2,2,2,2,2,2,2,2,2,2,2,2,2,2,2,2,2,2,2,2,2,2,2,2,2,2,2,2,2,2,2,2,2,2,2,2,2,2,2,2,2,2,2,2,2,2,2,2,2,2,2,2,2,2,2,2,2,2,2,2,2,2,2,2,2,2,2,2,2,2,2,2,2,2,2,2,2,2,2,2,2,2,2,2,2,2,2,2,2,2,2,2,2,2,2,2,2,2,2,2,2,2,2,2,2,2,2,2,2,2,2,2,2,2,2,2,2,2,2,2,2,2,2,2,2,2,2,2,2,2,2,2,2,2,2,2,2,2,2,2,2,2,2,2,2,2,2,2,2,2,2,2,2,2,2,2,2,2,2,2,2,2,2,2,2,2,2,2,2,2,2,2,2,2,2,2,2,2,2,2,2,2,2,2},'Factor',{1,1,1,1,1,1,1,1,1,1,1,1,1,1,1,1,1,1,1,1,1,1,1,1,1,1,1,1,1,1,1,1,1,1,1,1,1,1,1,1,1,1,1,1,1,1,1,1,1,1,1,1,1,1,1,1,1,1,1,1,1,1,1,1,1,1,1,1,1,1,1,1,1,1,1,1,1,1,1,1,1,1,1,1,1,1,1,1,1,1,1,1,1,1,1,1,1,1,1,1,1,1,1,1,1,1,1,1,1,1,1,1,1,1,1,1,1,1,1,1,1,1,1,1,1,1,1,1,1,1,1,1,1,1,1,1,1,1,1,1,1,1,1,1,1,1,1,1,1,1,1,1,1,1,1,1,1,1,1,1,1,1,1,1,1,1,1,1,1,1,1,1,1,1,1,1,1,1,1,1,1,1,1,1,1,1,1,1,1,1,1,1,1,1,1,1,1,1,1,1,1,1,1,1,1,1,1,1,1,1,1,1,1,1,1,1,1,1,1,1,1,1,1,1,1,1,1,1,1,1,1,1,1,1,1,1,1,1,1,1,1,1,1,1,1,1,1,1,1,1,1,1,1,1,1,1,1,1},'Offset',{-10,-10,-10,-10,-10,-10,-10,-10,-10,0,0,0,0,0,0,0,0,0,0,0,0,0,0,0,0,0,0,0,0,0,0,0,0,0,0,0,-10,-10,-10,-10,-10,-10,-10,-10,-10,0,0,0,0,0,0,0,0,0,0,0,0,0,0,0,0,0,0,0,0,0,0,0,0,0,0,0,-10,-10,-10,-10,-10,-10,-10,-10,-10,0,0,0,0,0,0,0,0,0,0,0,0,0,0,0,0,0,0,0,0,0,0,0,0,0,0,0,-10,-10,-10,-10,-10,-10,-10,-10,-10,0,0,0,0,0,0,0,0,0,0,0,0,0,0,0,0,0,0,0,0,0,0,0,0,0,0,0,-10,-10,-10,-10,-10,-10,-10,-10,-10,0,0,0,0,0,0,0,0,0,0,0,0,0,0,0,0,0,0,0,0,0,0,0,0,0,0,0,-10,-10,-10,-10,-10,-10,-10,-10,-10,0,0,0,0,0,0,0,0,0,0,0,0,0,0,0,0,0,0,0,0,0,0,0,0,0,0,0,-10,-10,-10,-10,-10,-10,-10,-10,-10,-10,0,0,0,0,0,0,0,0,0,0,0,0,0,0,0,0,0,0,0,0,0,0,0,0,0,0,0,0,0,0,0,0},'SgnComment',{'','','','','','','','','','','','','','','','','','','','','','','','','','','','','','','','','','','','','','','','','','','','','','','','','','','','','','','','','','','','','','','','','','','','','','','','','','','','','','','','','','','','','','','','','','','','','','','','','','','','','','','','','','','','','','','','','','','','','','','','','','','','','','','','','','','','','','','','','','','','','','','','','','','','','','','','','','','','','','','','','','','','','','','','','','','','','','','','','','','','','','','','','','','','','','','','','','','','','','','','','','','','','','','','','','','','','','','','','','','','','','','','','','','','','','','','','','','','','','','','','','','','','','','','','','','','','','','','','',''},'SgnUnit',{'dB','dB','dB','dB','dB','dB','dB','dB','dB','','','','','','','','','','','','','','','','','','','','','','','','','','','','dB','dB','dB','dB','dB','dB','dB','dB','dB','','','','','','','','','','','','','','','','','','','','','','','','','','','','dB','dB','dB','dB','dB','dB','dB','dB','dB','','','','','','','','','','','','','','','','','','','','','','','','','','','','dB','dB','dB','dB','dB','dB','dB','dB','dB','','','','','','','','','','','','','','','','','','','','','','','','','','','','dB','dB','dB','dB','dB','dB','dB','dB','dB','','','','','','','','','','','','','','','','','','','','','','','','','','','','dB','dB','dB','dB','dB','dB','dB','dB','dB','','','','','','','','','','','','','','','','','','','','','','','','','','','','dB','dB','dB','dB','dB','dB','dB','dB','dB','dB','','','','','','','','','','','','','','','','','','','','','','','','','','','','','','','',''},'Min',{-10,-10,-10,-10,-10,-10,-10,-10,-10,0,0,0,0,0,0,0,0,0,0,0,0,0,0,0,0,0,0,0,0,0,0,0,0,0,0,0,-10,-10,-10,-10,-10,-10,-10,-10,-10,0,0,0,0,0,0,0,0,0,0,0,0,0,0,0,0,0,0,0,0,0,0,0,0,0,0,0,-10,-10,-10,-10,-10,-10,-10,-10,-10,0,0,0,0,0,0,0,0,0,0,0,0,0,0,0,0,0,0,0,0,0,0,0,0,0,0,0,-10,-10,-10,-10,-10,-10,-10,-10,-10,0,0,0,0,0,0,0,0,0,0,0,0,0,0,0,0,0,0,0,0,0,0,0,0,0,0,0,-10,-10,-10,-10,-10,-10,-10,-10,-10,0,0,0,0,0,0,0,0,0,0,0,0,0,0,0,0,0,0,0,0,0,0,0,0,0,0,0,-10,-10,-10,-10,-10,-10,-10,-10,-10,0,0,0,0,0,0,0,0,0,0,0,0,0,0,0,0,0,0,0,0,0,0,0,0,0,0,0,-10,-10,-10,-10,-10,-10,-10,-10,-10,-10,0,0,0,0,0,0,0,0,0,0,0,0,0,0,0,0,0,0,0,0,0,0,0,0,0,0,0,0,0,0,0,0},'Max',{21,21,21,21,21,21,21,21,21,1,1,1,1,1,1,1,1,1,1,1,1,1,1,1,1,1,1,1,1,1,1,1,1,1,1,1,21,21,21,21,21,21,21,21,21,1,1,1,1,1,1,1,1,1,1,1,1,1,1,1,1,1,1,1,1,1,1,1,1,1,1,1,21,21,21,21,21,21,21,21,21,1,1,1,1,1,1,1,1,1,1,1,1,1,1,1,1,1,1,1,1,1,1,1,1,1,1,1,21,21,21,21,21,21,21,21,21,1,1,1,1,1,1,1,1,1,1,1,1,1,1,1,1,1,1,1,1,1,1,1,1,1,1,1,21,21,21,21,21,21,21,21,21,1,1,1,1,1,1,1,1,1,1,1,1,1,1,1,1,1,1,1,1,1,1,1,1,1,1,1,21,21,21,21,21,21,21,21,21,1,1,1,1,1,1,1,1,1,1,1,1,1,1,1,1,1,1,1,1,1,1,1,1,1,1,1,21,21,21,21,21,21,21,21,21,21,1,1,1,1,1,1,1,1,1,1,1,1,1,1,1,1,1,1,1,1,1,1,1,1,1,1,1,1,1,1,9,1},'SgnType',{2,2,2,2,2,2,2,2,2,2,2,2,2,2,2,2,2,2,2,2,2,2,2,2,2,2,2,2,2,2,2,2,2,2,2,2,2,2,2,2,2,2,2,2,2,2,2,2,2,2,2,2,2,2,2,2,2,2,2,2,2,2,2,2,2,2,2,2,2,2,2,2,2,2,2,2,2,2,2,2,2,2,2,2,2,2,2,2,2,2,2,2,2,2,2,2,2,2,2,2,2,2,2,2,2,2,2,2,2,2,2,2,2,2,2,2,2,2,2,2,2,2,2,2,2,2,2,2,2,2,2,2,2,2,2,2,2,2,2,2,2,2,2,2,2,2,2,2,2,2,2,2,2,2,2,2,2,2,2,2,2,2,2,2,2,2,2,2,2,2,2,2,2,2,2,2,2,2,2,2,2,2,2,2,2,2,2,2,2,2,2,2,2,2,2,2,2,2,2,2,2,2,2,2,2,2,2,2,2,2,2,2,2,2,2,2,2,2,2,2,2,2,2,2,2,2,2,2,2,2,2,2,2,2,2,2,2,2,2,2,2,2,2,2,2,2,2,2,2,2,2,2,2,2,2,2,1,0},'SLDataType',{'SS_DOUBLE','SS_DOUBLE','SS_DOUBLE','SS_DOUBLE','SS_DOUBLE','SS_DOUBLE','SS_DOUBLE','SS_DOUBLE','SS_DOUBLE','SS_DOUBLE','SS_DOUBLE','SS_DOUBLE','SS_DOUBLE','SS_DOUBLE','SS_DOUBLE','SS_DOUBLE','SS_DOUBLE','SS_DOUBLE','SS_DOUBLE','SS_DOUBLE','SS_DOUBLE','SS_DOUBLE','SS_DOUBLE','SS_DOUBLE','SS_DOUBLE','SS_DOUBLE','SS_DOUBLE','SS_DOUBLE','SS_DOUBLE','SS_DOUBLE','SS_DOUBLE','SS_DOUBLE','SS_DOUBLE','SS_DOUBLE','SS_DOUBLE','SS_DOUBLE','SS_DOUBLE','SS_DOUBLE','SS_DOUBLE','SS_DOUBLE','SS_DOUBLE','SS_DOUBLE','SS_DOUBLE','SS_DOUBLE','SS_DOUBLE','SS_DOUBLE','SS_DOUBLE','SS_DOUBLE','SS_DOUBLE','SS_DOUBLE','SS_DOUBLE','SS_DOUBLE','SS_DOUBLE','SS_DOUBLE','SS_DOUBLE','SS_DOUBLE','SS_DOUBLE','SS_DOUBLE','SS_DOUBLE','SS_DOUBLE','SS_DOUBLE','SS_DOUBLE','SS_DOUBLE','SS_DOUBLE','SS_DOUBLE','SS_DOUBLE','SS_DOUBLE','SS_DOUBLE','SS_DOUBLE','SS_DOUBLE','SS_DOUBLE','SS_DOUBLE','SS_DOUBLE','SS_DOUBLE','SS_DOUBLE','SS_DOUBLE','SS_DOUBLE','SS_DOUBLE','SS_DOUBLE','SS_DOUBLE','SS_DOUBLE','SS_DOUBLE','SS_DOUBLE','SS_DOUBLE','SS_DOUBLE','SS_DOUBLE','SS_DOUBLE','SS_DOUBLE','SS_DOUBLE','SS_DOUBLE','SS_DOUBLE','SS_DOUBLE','SS_DOUBLE','SS_DOUBLE','SS_DOUBLE','SS_DOUBLE','SS_DOUBLE','SS_DOUBLE','SS_DOUBLE','SS_DOUBLE','SS_DOUBLE','SS_DOUBLE','SS_DOUBLE','SS_DOUBLE','SS_DOUBLE','SS_DOUBLE','SS_DOUBLE','SS_DOUBLE','SS_DOUBLE','SS_DOUBLE','SS_DOUBLE','SS_DOUBLE','SS_DOUBLE','SS_DOUBLE','SS_DOUBLE','SS_DOUBLE','SS_DOUBLE','SS_DOUBLE','SS_DOUBLE','SS_DOUBLE','SS_DOUBLE','SS_DOUBLE','SS_DOUBLE','SS_DOUBLE','SS_DOUBLE','SS_DOUBLE','SS_DOUBLE','SS_DOUBLE','SS_DOUBLE','SS_DOUBLE','SS_DOUBLE','SS_DOUBLE','SS_DOUBLE','SS_DOUBLE','SS_DOUBLE','SS_DOUBLE','SS_DOUBLE','SS_DOUBLE','SS_DOUBLE','SS_DOUBLE','SS_DOUBLE','SS_DOUBLE','SS_DOUBLE','SS_DOUBLE','SS_DOUBLE','SS_DOUBLE','SS_DOUBLE','SS_DOUBLE','SS_DOUBLE','SS_DOUBLE','SS_DOUBLE','SS_DOUBLE','SS_DOUBLE','SS_DOUBLE','SS_DOUBLE','SS_DOUBLE','SS_DOUBLE','SS_DOUBLE','SS_DOUBLE','SS_DOUBLE','SS_DOUBLE','SS_DOUBLE','SS_DOUBLE','SS_DOUBLE','SS_DOUBLE','SS_DOUBLE','SS_DOUBLE','SS_DOUBLE','SS_DOUBLE','SS_DOUBLE','SS_DOUBLE','SS_DOUBLE','SS_DOUBLE','SS_DOUBLE','SS_DOUBLE','SS_DOUBLE','SS_DOUBLE','SS_DOUBLE','SS_DOUBLE','SS_DOUBLE','SS_DOUBLE','SS_DOUBLE','SS_DOUBLE','SS_DOUBLE','SS_DOUBLE','SS_DOUBLE','SS_DOUBLE','SS_DOUBLE','SS_DOUBLE','SS_DOUBLE','SS_DOUBLE','SS_DOUBLE','SS_DOUBLE','SS_DOUBLE','SS_DOUBLE','SS_DOUBLE','SS_DOUBLE','SS_DOUBLE','SS_DOUBLE','SS_DOUBLE','SS_DOUBLE','SS_DOUBLE','SS_DOUBLE','SS_DOUBLE','SS_DOUBLE','SS_DOUBLE','SS_DOUBLE','SS_DOUBLE','SS_DOUBLE','SS_DOUBLE','SS_DOUBLE','SS_DOUBLE','SS_DOUBLE','SS_DOUBLE','SS_DOUBLE','SS_DOUBLE','SS_DOUBLE','SS_DOUBLE','SS_DOUBLE','SS_DOUBLE','SS_DOUBLE','SS_DOUBLE','SS_DOUBLE','SS_DOUBLE','SS_DOUBLE','SS_DOUBLE','SS_DOUBLE','SS_DOUBLE','SS_DOUBLE','SS_DOUBLE','SS_DOUBLE','SS_DOUBLE','SS_DOUBLE','SS_DOUBLE','SS_DOUBLE','SS_DOUBLE','SS_DOUBLE','SS_DOUBLE','SS_DOUBLE','SS_DOUBLE','SS_DOUBLE','SS_DOUBLE','SS_DOUBLE','SS_DOUBLE','SS_DOUBLE','SS_DOUBLE','SS_DOUBLE','SS_DOUBLE','SS_DOUBLE','SS_DOUBLE','SS_DOUBLE','SS_DOUBLE','SS_DOUBLE','SS_DOUBLE','SS_DOUBLE','SS_DOUBLE','SS_DOUBLE','SS_DOUBLE'},'DataType',{0,0,0,0,0,0,0,0,0,0,0,0,0,0,0,0,0,0,0,0,0,0,0,0,0,0,0,0,0,0,0,0,0,0,0,0,0,0,0,0,0,0,0,0,0,0,0,0,0,0,0,0,0,0,0,0,0,0,0,0,0,0,0,0,0,0,0,0,0,0,0,0,0,0,0,0,0,0,0,0,0,0,0,0,0,0,0,0,0,0,0,0,0,0,0,0,0,0,0,0,0,0,0,0,0,0,0,0,0,0,0,0,0,0,0,0,0,0,0,0,0,0,0,0,0,0,0,0,0,0,0,0,0,0,0,0,0,0,0,0,0,0,0,0,0,0,0,0,0,0,0,0,0,0,0,0,0,0,0,0,0,0,0,0,0,0,0,0,0,0,0,0,0,0,0,0,0,0,0,0,0,0,0,0,0,0,0,0,0,0,0,0,0,0,0,0,0,0,0,0,0,0,0,0,0,0,0,0,0,0,0,0,0,0,0,0,0,0,0,0,0,0,0,0,0,0,0,0,0,0,0,0,0,0,0,0,0,0,0,0,0,0,0,0,0,0,0,0,0,0,0,0,0,0,0,0,0,0},'ModeValue',{0,1,2,3,4,5,6,7,8,0,1,2,3,4,5,6,7,8,0,1,2,3,4,5,6,7,8,0,1,2,3,4,5,6,7,8,0,1,2,3,4,5,6,7,8,0,1,2,3,4,5,6,7,8,0,1,2,3,4,5,6,7,8,0,1,2,3,4,5,6,7,8,0,1,2,3,4,5,6,7,8,0,1,2,3,4,5,6,7,8,0,1,2,3,4,5,6,7,8,0,1,2,3,4,5,6,7,8,0,1,2,3,4,5,6,7,8,0,1,2,3,4,5,6,7,8,0,1,2,3,4,5,6,7,8,0,1,2,3,4,5,6,7,8,0,1,2,3,4,5,6,7,8,0,1,2,3,4,5,6,7,8,0,1,2,3,4,5,6,7,8,0,1,2,3,4,5,6,7,8,0,1,2,3,4,5,6,7,8,0,1,2,3,4,5,6,7,8,0,1,2,3,4,5,6,7,8,0,1,2,3,4,5,6,7,8,0,1,2,3,4,5,6,7,8,9,0,1,2,3,4,5,6,7,8,9,0,1,2,3,4,5,6,7,8,9,0,1,2,3,4,5,6,7,8,9,-1,-1}),'MsgIdNumFormat',0,'MsgComment',{{''}}),'Version',1.2,'general',struct('isFromLib',0)),'OFF',[]}},'GroupId',{{struct('Group',{{'RTICAN'}},'No',4,'Behavior',{{'NAMECHANGE'}},'BlockType',{{'SINK'}},'NameChangeFlag',0),'OFF',[]}},'SFcnRTICANMessage',{{struct('MsgType','RX','SFcnPortType','Scalar','MsgName','ESR_TrackMotionPower','MsgIdFormat','STD','MsgId',1344,'MsgLength',8,'NumSignals',258,'SampleTime',0.01,'Signal',struct('SgnName',{'CAN_TX_TRACK_POWER07','CAN_TX_TRACK_POWER14','CAN_TX_TRACK_POWER21','CAN_TX_TRACK_POWER28','CAN_TX_TRACK_POWER35','CAN_TX_TRACK_POWER42','CAN_TX_TRACK_POWER49','CAN_TX_TRACK_POWER56','CAN_TX_TRACK_POWER63','CAN_TX_TRACK_MOVING07','CAN_TX_TRACK_MOVING14','CAN_TX_TRACK_MOVING21','CAN_TX_TRACK_MOVING28','CAN_TX_TRACK_MOVING35','CAN_TX_TRACK_MOVING42','CAN_TX_TRACK_MOVING49','CAN_TX_TRACK_MOVING56','CAN_TX_TRACK_MOVING63','CAN_TX_TRACK_MOVABLE_SLOW07','CAN_TX_TRACK_MOVABLE_SLOW14','CAN_TX_TRACK_MOVABLE_SLOW21','CAN_TX_TRACK_MOVABLE_SLOW28','CAN_TX_TRACK_MOVABLE_SLOW35','CAN_TX_TRACK_MOVABLE_SLOW42','CAN_TX_TRACK_MOVABLE_SLOW49','CAN_TX_TRACK_MOVABLE_SLOW56','CAN_TX_TRACK_MOVABLE_SLOW63','CAN_TX_TRACK_MOVABLE_FAST07','CAN_TX_TRACK_MOVABLE_FAST14','CAN_TX_TRACK_MOVABLE_FAST21','CAN_TX_TRACK_MOVABLE_FAST28','CAN_TX_TRACK_MOVABLE_FAST35','CAN_TX_TRACK_MOVABLE_FAST42','CAN_TX_TRACK_MOVABLE_FAST49','CAN_TX_TRACK_MOVABLE_FAST56','CAN_TX_TRACK_MOVABLE_FAST63','CAN_TX_TRACK_POWER06','CAN_TX_TRACK_POWER13','CAN_TX_TRACK_POWER20','CAN_TX_TRACK_POWER27','CAN_TX_TRACK_POWER34','CAN_TX_TRACK_POWER41','CAN_TX_TRACK_POWER48','CAN_TX_TRACK_POWER55','CAN_TX_TRACK_POWER62','CAN_TX_TRACK_MOVING06','CAN_TX_TRACK_MOVING13','CAN_TX_TRACK_MOVING20','CAN_TX_TRACK_MOVING27','CAN_TX_TRACK_MOVING34','CAN_TX_TRACK_MOVING41','CAN_TX_TRACK_MOVING48','CAN_TX_TRACK_MOVING55','CAN_TX_TRACK_MOVING62','CAN_TX_TRACK_MOVABLE_SLOW06','CAN_TX_TRACK_MOVABLE_SLOW13','CAN_TX_TRACK_MOVABLE_SLOW20','CAN_TX_TRACK_MOVABLE_SLOW27','CAN_TX_TRACK_MOVABLE_SLOW34','CAN_TX_TRACK_MOVABLE_SLOW41','CAN_TX_TRACK_MOVABLE_SLOW48','CAN_TX_TRACK_MOVABLE_SLOW55','CAN_TX_TRACK_MOVABLE_SLOW62','CAN_TX_TRACK_MOVABLE_FAST06','CAN_TX_TRACK_MOVABLE_FAST13','CAN_TX_TRACK_MOVABLE_FAST20','CAN_TX_TRACK_MOVABLE_FAST27','CAN_TX_TRACK_MOVABLE_FAST34','CAN_TX_TRACK_MOVABLE_FAST41','CAN_TX_TRACK_MOVABLE_FAST48','CAN_TX_TRACK_MOVABLE_FAST55','CAN_TX_TRACK_MOVABLE_FAST62','CAN_TX_TRACK_POWER05','CAN_TX_TRACK_POWER12','CAN_TX_TRACK_POWER19','CAN_TX_TRACK_POWER26','CAN_TX_TRACK_POWER33','CAN_TX_TRACK_POWER40','CAN_TX_TRACK_POWER47','CAN_TX_TRACK_POWER54','CAN_TX_TRACK_POWER61','CAN_TX_TRACK_MOVING05','CAN_TX_TRACK_MOVING12','CAN_TX_TRACK_MOVING19','CAN_TX_TRACK_MOVING26','CAN_TX_TRACK_MOVING33','CAN_TX_TRACK_MOVING40','CAN_TX_TRACK_MOVING47','CAN_TX_TRACK_MOVING54','CAN_TX_TRACK_MOVING61','CAN_TX_TRACK_MOVABLE_SLOW05','CAN_TX_TRACK_MOVABLE_SLOW12','CAN_TX_TRACK_MOVABLE_SLOW19','CAN_TX_TRACK_MOVABLE_SLOW26','CAN_TX_TRACK_MOVABLE_SLOW33','CAN_TX_TRACK_MOVABLE_SLOW40','CAN_TX_TRACK_MOVABLE_SLOW47','CAN_TX_TRACK_MOVABLE_SLOW54','CAN_TX_TRACK_MOVABLE_SLOW61','CAN_TX_TRACK_MOVABLE_FAST05','CAN_TX_TRACK_MOVABLE_FAST12','CAN_TX_TRACK_MOVABLE_FAST19','CAN_TX_TRACK_MOVABLE_FAST26','CAN_TX_TRACK_MOVABLE_FAST33','CAN_TX_TRACK_MOVABLE_FAST40','CAN_TX_TRACK_MOVABLE_FAST47','CAN_TX_TRACK_MOVABLE_FAST54','CAN_TX_TRACK_MOVABLE_FAST61','CAN_TX_TRACK_POWER04','CAN_TX_TRACK_POWER11','CAN_TX_TRACK_POWER18','CAN_TX_TRACK_POWER25','CAN_TX_TRACK_POWER32','CAN_TX_TRACK_POWER39','CAN_TX_TRACK_POWER46','CAN_TX_TRACK_POWER53','CAN_TX_TRACK_POWER60','CAN_TX_TRACK_MOVING04','CAN_TX_TRACK_MOVING11','CAN_TX_TRACK_MOVING18','CAN_TX_TRACK_MOVING25','CAN_TX_TRACK_MOVING32','CAN_TX_TRACK_MOVING39','CAN_TX_TRACK_MOVING46','CAN_TX_TRACK_MOVING53','CAN_TX_TRACK_MOVING60','CAN_TX_TRACK_MOVABLE_SLOW04','CAN_TX_TRACK_MOVABLE_SLOW11','CAN_TX_TRACK_MOVABLE_SLOW18','CAN_TX_TRACK_MOVABLE_SLOW25','CAN_TX_TRACK_MOVABLE_SLOW32','CAN_TX_TRACK_MOVABLE_SLOW39','CAN_TX_TRACK_MOVABLE_SLOW46','CAN_TX_TRACK_MOVABLE_SLOW53','CAN_TX_TRACK_MOVABLE_SLOW60','CAN_TX_TRACK_MOVABLE_FAST04','CAN_TX_TRACK_MOVABLE_FAST11','CAN_TX_TRACK_MOVABLE_FAST18','CAN_TX_TRACK_MOVABLE_FAST25','CAN_TX_TRACK_MOVABLE_FAST32','CAN_TX_TRACK_MOVABLE_FAST39','CAN_TX_TRACK_MOVABLE_FAST46','CAN_TX_TRACK_MOVABLE_FAST53','CAN_TX_TRACK_MOVABLE_FAST60','CAN_TX_TRACK_POWER03','CAN_TX_TRACK_POWER10','CAN_TX_TRACK_POWER17','CAN_TX_TRACK_POWER24','CAN_TX_TRACK_POWER31','CAN_TX_TRACK_POWER38','CAN_TX_TRACK_POWER45','CAN_TX_TRACK_POWER52','CAN_TX_TRACK_POWER59','CAN_TX_TRACK_MOVING03','CAN_TX_TRACK_MOVING10','CAN_TX_TRACK_MOVING17','CAN_TX_TRACK_MOVING24','CAN_TX_TRACK_MOVING31','CAN_TX_TRACK_MOVING38','CAN_TX_TRACK_MOVING45','CAN_TX_TRACK_MOVING52','CAN_TX_TRACK_MOVING59','CAN_TX_TRACK_MOVABLE_SLOW03','CAN_TX_TRACK_MOVABLE_SLOW10','CAN_TX_TRACK_MOVABLE_SLOW17','CAN_TX_TRACK_MOVABLE_SLOW24','CAN_TX_TRACK_MOVABLE_SLOW31','CAN_TX_TRACK_MOVABLE_SLOW38','CAN_TX_TRACK_MOVABLE_SLOW45','CAN_TX_TRACK_MOVABLE_SLOW52','CAN_TX_TRACK_MOVABLE_SLOW59','CAN_TX_TRACK_MOVABLE_FAST03','CAN_TX_TRACK_MOVABLE_FAST10','CAN_TX_TRACK_MOVABLE_FAST17','CAN_TX_TRACK_MOVABLE_FAST24','CAN_TX_TRACK_MOVABLE_FAST31','CAN_TX_TRACK_MOVABLE_FAST38','CAN_TX_TRACK_MOVABLE_FAST45','CAN_TX_TRACK_MOVABLE_FAST52','CAN_TX_TRACK_MOVABLE_FAST59','CAN_TX_TRACK_POWER02','CAN_TX_TRACK_POWER09','CAN_TX_TRACK_POWER16','CAN_TX_TRACK_POWER23','CAN_TX_TRACK_POWER30','CAN_TX_TRACK_POWER37','CAN_TX_TRACK_POWER44','CAN_TX_TRACK_POWER51','CAN_TX_TRACK_POWER58','CAN_TX_TRACK_MOVING02','CAN_TX_TRACK_MOVING09','CAN_TX_TRACK_MOVING16','CAN_TX_TRACK_MOVING23','CAN_TX_TRACK_MOVING30','CAN_TX_TRACK_MOVING37','CAN_TX_TRACK_MOVING44','CAN_TX_TRACK_MOVING51','CAN_TX_TRACK_MOVING58','CAN_TX_TRACK_MOVABLE_SLOW02','CAN_TX_TRACK_MOVABLE_SLOW09','CAN_TX_TRACK_MOVABLE_SLOW16','CAN_TX_TRACK_MOVABLE_SLOW23','CAN_TX_TRACK_MOVABLE_SLOW30','CAN_TX_TRACK_MOVABLE_SLOW37','CAN_TX_TRACK_MOVABLE_SLOW44','CAN_TX_TRACK_MOVABLE_SLOW51','CAN_TX_TRACK_MOVABLE_SLOW58','CAN_TX_TRACK_MOVABLE_FAST02','CAN_TX_TRACK_MOVABLE_FAST09','CAN_TX_TRACK_MOVABLE_FAST16','CAN_TX_TRACK_MOVABLE_FAST23','CAN_TX_TRACK_MOVABLE_FAST30','CAN_TX_TRACK_MOVABLE_FAST37','CAN_TX_TRACK_MOVABLE_FAST44','CAN_TX_TRACK_MOVABLE_FAST51','CAN_TX_TRACK_MOVABLE_FAST58','CAN_TX_TRACK_POWER01','CAN_TX_TRACK_POWER08','CAN_TX_TRACK_POWER15','CAN_TX_TRACK_POWER22','CAN_TX_TRACK_POWER29','CAN_TX_TRACK_POWER36','CAN_TX_TRACK_POWER43','CAN_TX_TRACK_POWER50','CAN_TX_TRACK_POWER57','CAN_TX_TRACK_POWER64','CAN_TX_TRACK_MOVING01','CAN_TX_TRACK_MOVING08','CAN_TX_TRACK_MOVING15','CAN_TX_TRACK_MOVING22','CAN_TX_TRACK_MOVING29','CAN_TX_TRACK_MOVING36','CAN_TX_TRACK_MOVING43','CAN_TX_TRACK_MOVING50','CAN_TX_TRACK_MOVING57','CAN_TX_TRACK_MOVING64','CAN_TX_TRACK_MOVABLE_SLOW01','CAN_TX_TRACK_MOVABLE_SLOW08','CAN_TX_TRACK_MOVABLE_SLOW15','CAN_TX_TRACK_MOVABLE_SLOW22','CAN_TX_TRACK_MOVABLE_SLOW29','CAN_TX_TRACK_MOVABLE_SLOW36','CAN_TX_TRACK_MOVABLE_SLOW43','CAN_TX_TRACK_MOVABLE_SLOW50','CAN_TX_TRACK_MOVABLE_SLOW57','CAN_TX_TRACK_MOVABLE_SLOW64','CAN_TX_TRACK_MOVABLE_FAST01','CAN_TX_TRACK_MOVABLE_FAST08','CAN_TX_TRACK_MOVABLE_FAST15','CAN_TX_TRACK_MOVABLE_FAST22','CAN_TX_TRACK_MOVABLE_FAST29','CAN_TX_TRACK_MOVABLE_FAST36','CAN_TX_TRACK_MOVABLE_FAST43','CAN_TX_TRACK_MOVABLE_FAST50','CAN_TX_TRACK_MOVABLE_FAST57','CAN_TX_TRACK_MOVABLE_FAST64','CAN_TX_TRACK_CAN_ID_GROUP','CAN_TX_TRACK_ROLLING_COUNT_2'},'SgnStartBit',{0,0,0,0,0,0,0,0,0,5,5,5,5,5,5,5,5,5,6,6,6,6,6,6,6,6,6,7,7,7,7,7,7,7,7,7,8,8,8,8,8,8,8,8,8,13,13,13,13,13,13,13,13,13,14,14,14,14,14,14,14,14,14,15,15,15,15,15,15,15,15,15,16,16,16,16,16,16,16,16,16,21,21,21,21,21,21,21,21,21,22,22,22,22,22,22,22,22,22,23,23,23,23,23,23,23,23,23,24,24,24,24,24,24,24,24,24,29,29,29,29,29,29,29,29,29,30,30,30,30,30,30,30,30,30,31,31,31,31,31,31,31,31,31,32,32,32,32,32,32,32,32,32,37,37,37,37,37,37,37,37,37,38,38,38,38,38,38,38,38,38,39,39,39,39,39,39,39,39,39,40,40,40,40,40,40,40,40,40,45,45,45,45,45,45,45,45,45,46,46,46,46,46,46,46,46,46,47,47,47,47,47,47,47,47,47,48,48,48,48,48,48,48,48,48,48,53,53,53,53,53,53,53,53,53,53,54,54,54,54,54,54,54,54,54,54,55,55,55,55,55,55,55,55,55,55,56,60},'SgnLength',{5,5,5,5,5,5,5,5,5,1,1,1,1,1,1,1,1,1,1,1,1,1,1,1,1,1,1,1,1,1,1,1,1,1,1,1,5,5,5,5,5,5,5,5,5,1,1,1,1,1,1,1,1,1,1,1,1,1,1,1,1,1,1,1,1,1,1,1,1,1,1,1,5,5,5,5,5,5,5,5,5,1,1,1,1,1,1,1,1,1,1,1,1,1,1,1,1,1,1,1,1,1,1,1,1,1,1,1,5,5,5,5,5,5,5,5,5,1,1,1,1,1,1,1,1,1,1,1,1,1,1,1,1,1,1,1,1,1,1,1,1,1,1,1,5,5,5,5,5,5,5,5,5,1,1,1,1,1,1,1,1,1,1,1,1,1,1,1,1,1,1,1,1,1,1,1,1,1,1,1,5,5,5,5,5,5,5,5,5,1,1,1,1,1,1,1,1,1,1,1,1,1,1,1,1,1,1,1,1,1,1,1,1,1,1,1,5,5,5,5,5,5,5,5,5,5,1,1,1,1,1,1,1,1,1,1,1,1,1,1,1,1,1,1,1,1,1,1,1,1,1,1,1,1,1,1,4,1},'ByteLayout',{['motorola back.'],['motorola back.'],['motorola back.'],['motorola back.'],['motorola back.'],['motorola back.'],['motorola back.'],['motorola back.'],['motorola back.'],['motorola back.'],['motorola back.'],['motorola back.'],['motorola back.'],['motorola back.'],['motorola back.'],['motorola back.'],['motorola back.'],['motorola back.'],['motorola back.'],['motorola back.'],['motorola back.'],['motorola back.'],['motorola back.'],['motorola back.'],['motorola back.'],['motorola back.'],['motorola back.'],['motorola back.'],['motorola back.'],['motorola back.'],['motorola back.'],['motorola back.'],['motorola back.'],['motorola back.'],['motorola back.'],['motorola back.'],['motorola back.'],['motorola back.'],['motorola back.'],['motorola back.'],['motorola back.'],['motorola back.'],['motorola back.'],['motorola back.'],['motorola back.'],['motorola back.'],['motorola back.'],['motorola back.'],['motorola back.'],['motorola back.'],['motorola back.'],['motorola back.'],['motorola back.'],['motorola back.'],['motorola back.'],['motorola back.'],['motorola back.'],['motorola back.'],['motorola back.'],['motorola back.'],['motorola back.'],['motorola back.'],['motorola back.'],['motorola back.'],['motorola back.'],['motorola back.'],['motorola back.'],['motorola back.'],['motorola back.'],['motorola back.'],['motorola back.'],['motorola back.'],['motorola back.'],['motorola back.'],['motorola back.'],['motorola back.'],['motorola back.'],['motorola back.'],['motorola back.'],['motorola back.'],['motorola back.'],['motorola back.'],['motorola back.'],['motorola back.'],['motorola back.'],['motorola back.'],['motorola back.'],['motorola back.'],['motorola back.'],['motorola back.'],['motorola back.'],['motorola back.'],['motorola back.'],['motorola back.'],['motorola back.'],['motorola back.'],['motorola back.'],['motorola back.'],['motorola back.'],['motorola back.'],['motorola back.'],['motorola back.'],['motorola back.'],['motorola back.'],['motorola back.'],['motorola back.'],['motorola back.'],['motorola back.'],['motorola back.'],['motorola back.'],['motorola back.'],['motorola back.'],['motorola back.'],['motorola back.'],['motorola back.'],['motorola back.'],['motorola back.'],['motorola back.'],['motorola back.'],['motorola back.'],['motorola back.'],['motorola back.'],['motorola back.'],['motorola back.'],['motorola back.'],['motorola back.'],['motorola back.'],['motorola back.'],['motorola back.'],['motorola back.'],['motorola back.'],['motorola back.'],['motorola back.'],['motorola back.'],['motorola back.'],['motorola back.'],['motorola back.'],['motorola back.'],['motorola back.'],['motorola back.'],['motorola back.'],['motorola back.'],['motorola back.'],['motorola back.'],['motorola back.'],['motorola back.'],['motorola back.'],['motorola back.'],['motorola back.'],['motorola back.'],['motorola back.'],['motorola back.'],['motorola back.'],['motorola back.'],['motorola back.'],['motorola back.'],['motorola back.'],['motorola back.'],['motorola back.'],['motorola back.'],['motorola back.'],['motorola back.'],['motorola back.'],['motorola back.'],['motorola back.'],['motorola back.'],['motorola back.'],['motorola back.'],['motorola back.'],['motorola back.'],['motorola back.'],['motorola back.'],['motorola back.'],['motorola back.'],['motorola back.'],['motorola back.'],['motorola back.'],['motorola back.'],['motorola back.'],['motorola back.'],['motorola back.'],['motorola back.'],['motorola back.'],['motorola back.'],['motorola back.'],['motorola back.'],['motorola back.'],['motorola back.'],['motorola back.'],['motorola back.'],['motorola back.'],['motorola back.'],['motorola back.'],['motorola back.'],['motorola back.'],['motorola back.'],['motorola back.'],['motorola back.'],['motorola back.'],['motorola back.'],['motorola back.'],['motorola back.'],['motorola back.'],['motorola back.'],['motorola back.'],['motorola back.'],['motorola back.'],['motorola back.'],['motorola back.'],['motorola back.'],['motorola back.'],['motorola back.'],['motorola back.'],['motorola back.'],['motorola back.'],['motorola back.'],['motorola back.'],['motorola back.'],['motorola back.'],['motorola back.'],['motorola back.'],['motorola back.'],['motorola back.'],['motorola back.'],['motorola back.'],['motorola back.'],['motorola back.'],['motorola back.'],['motorola back.'],['motorola back.'],['motorola back.'],['motorola back.'],['motorola back.'],['motorola back.'],['motorola back.'],['motorola back.'],['motorola back.'],['motorola back.'],['motorola back.'],['motorola back.'],['motorola back.'],['motorola back.'],['motorola back.'],['motorola back.'],['motorola back.'],['motorola back.'],['motorola back.'],['motorola back.'],['motorola back.'],['motorola back.'],['motorola back.'],['motorola back.'],['motorola back.'],['motorola back.'],['motorola back.'],['motorola back.'],['motorola back.'],['motorola back.']},'Factor',{1,1,1,1,1,1,1,1,1,1,1,1,1,1,1,1,1,1,1,1,1,1,1,1,1,1,1,1,1,1,1,1,1,1,1,1,1,1,1,1,1,1,1,1,1,1,1,1,1,1,1,1,1,1,1,1,1,1,1,1,1,1,1,1,1,1,1,1,1,1,1,1,1,1,1,1,1,1,1,1,1,1,1,1,1,1,1,1,1,1,1,1,1,1,1,1,1,1,1,1,1,1,1,1,1,1,1,1,1,1,1,1,1,1,1,1,1,1,1,1,1,1,1,1,1,1,1,1,1,1,1,1,1,1,1,1,1,1,1,1,1,1,1,1,1,1,1,1,1,1,1,1,1,1,1,1,1,1,1,1,1,1,1,1,1,1,1,1,1,1,1,1,1,1,1,1,1,1,1,1,1,1,1,1,1,1,1,1,1,1,1,1,1,1,1,1,1,1,1,1,1,1,1,1,1,1,1,1,1,1,1,1,1,1,1,1,1,1,1,1,1,1,1,1,1,1,1,1,1,1,1,1,1,1,1,1,1,1,1,1,1,1,1,1,1,1,1,1,1,1,1,1,1,1,1,1,1,1},'Offset',{-10,-10,-10,-10,-10,-10,-10,-10,-10,0,0,0,0,0,0,0,0,0,0,0,0,0,0,0,0,0,0,0,0,0,0,0,0,0,0,0,-10,-10,-10,-10,-10,-10,-10,-10,-10,0,0,0,0,0,0,0,0,0,0,0,0,0,0,0,0,0,0,0,0,0,0,0,0,0,0,0,-10,-10,-10,-10,-10,-10,-10,-10,-10,0,0,0,0,0,0,0,0,0,0,0,0,0,0,0,0,0,0,0,0,0,0,0,0,0,0,0,-10,-10,-10,-10,-10,-10,-10,-10,-10,0,0,0,0,0,0,0,0,0,0,0,0,0,0,0,0,0,0,0,0,0,0,0,0,0,0,0,-10,-10,-10,-10,-10,-10,-10,-10,-10,0,0,0,0,0,0,0,0,0,0,0,0,0,0,0,0,0,0,0,0,0,0,0,0,0,0,0,-10,-10,-10,-10,-10,-10,-10,-10,-10,0,0,0,0,0,0,0,0,0,0,0,0,0,0,0,0,0,0,0,0,0,0,0,0,0,0,0,-10,-10,-10,-10,-10,-10,-10,-10,-10,-10,0,0,0,0,0,0,0,0,0,0,0,0,0,0,0,0,0,0,0,0,0,0,0,0,0,0,0,0,0,0,0,0},'SgnType',{'mode-dependent','mode-dependent','mode-dependent','mode-dependent','mode-dependent','mode-dependent','mode-dependent','mode-dependent','mode-dependent','mode-dependent','mode-dependent','mode-dependent','mode-dependent','mode-dependent','mode-dependent','mode-dependent','mode-dependent','mode-dependent','mode-dependent','mode-dependent','mode-dependent','mode-dependent','mode-dependent','mode-dependent','mode-dependent','mode-dependent','mode-dependent','mode-dependent','mode-dependent','mode-dependent','mode-dependent','mode-dependent','mode-dependent','mode-dependent','mode-dependent','mode-dependent','mode-dependent','mode-dependent','mode-dependent','mode-dependent','mode-dependent','mode-dependent','mode-dependent','mode-dependent','mode-dependent','mode-dependent','mode-dependent','mode-dependent','mode-dependent','mode-dependent','mode-dependent','mode-dependent','mode-dependent','mode-dependent','mode-dependent','mode-dependent','mode-dependent','mode-dependent','mode-dependent','mode-dependent','mode-dependent','mode-dependent','mode-dependent','mode-dependent','mode-dependent','mode-dependent','mode-dependent','mode-dependent','mode-dependent','mode-dependent','mode-dependent','mode-dependent','mode-dependent','mode-dependent','mode-dependent','mode-dependent','mode-dependent','mode-dependent','mode-dependent','mode-dependent','mode-dependent','mode-dependent','mode-dependent','mode-dependent','mode-dependent','mode-dependent','mode-dependent','mode-dependent','mode-dependent','mode-dependent','mode-dependent','mode-dependent','mode-dependent','mode-dependent','mode-dependent','mode-dependent','mode-dependent','mode-dependent','mode-dependent','mode-dependent','mode-dependent','mode-dependent','mode-dependent','mode-dependent','mode-dependent','mode-dependent','mode-dependent','mode-dependent','mode-dependent','mode-dependent','mode-dependent','mode-dependent','mode-dependent','mode-dependent','mode-dependent','mode-dependent','mode-dependent','mode-dependent','mode-dependent','mode-dependent','mode-dependent','mode-dependent','mode-dependent','mode-dependent','mode-dependent','mode-dependent','mode-dependent','mode-dependent','mode-dependent','mode-dependent','mode-dependent','mode-dependent','mode-dependent','mode-dependent','mode-dependent','mode-dependent','mode-dependent','mode-dependent','mode-dependent','mode-dependent','mode-dependent','mode-dependent','mode-dependent','mode-dependent','mode-dependent','mode-dependent','mode-dependent','mode-dependent','mode-dependent','mode-dependent','mode-dependent','mode-dependent','mode-dependent','mode-dependent','mode-dependent','mode-dependent','mode-dependent','mode-dependent','mode-dependent','mode-dependent','mode-dependent','mode-dependent','mode-dependent','mode-dependent','mode-dependent','mode-dependent','mode-dependent','mode-dependent','mode-dependent','mode-dependent','mode-dependent','mode-dependent','mode-dependent','mode-dependent','mode-dependent','mode-dependent','mode-dependent','mode-dependent','mode-dependent','mode-dependent','mode-dependent','mode-dependent','mode-dependent','mode-dependent','mode-dependent','mode-dependent','mode-dependent','mode-dependent','mode-dependent','mode-dependent','mode-dependent','mode-dependent','mode-dependent','mode-dependent','mode-dependent','mode-dependent','mode-dependent','mode-dependent','mode-dependent','mode-dependent','mode-dependent','mode-dependent','mode-dependent','mode-dependent','mode-dependent','mode-dependent','mode-dependent','mode-dependent','mode-dependent','mode-dependent','mode-dependent','mode-dependent','mode-dependent','mode-dependent','mode-dependent','mode-dependent','mode-dependent','mode-dependent','mode-dependent','mode-dependent','mode-dependent','mode-dependent','mode-dependent','mode-dependent','mode-dependent','mode-dependent','mode-dependent','mode-dependent','mode-dependent','mode-dependent','mode-dependent','mode-dependent','mode-dependent','mode-dependent','mode-dependent','mode-dependent','mode-dependent','mode-dependent','mode-dependent','mode-dependent','mode-dependent','mode-dependent','mode-dependent','mode-dependent','mode-dependent','mode-dependent','mode-dependent','mode-dependent','mode-dependent','mode-dependent','mode-dependent','mode-dependent','mode-dependent','mode-dependent','mode-dependent','mode-dependent','mode','standard'},'SLDataType',{'SS_DOUBLE','SS_DOUBLE','SS_DOUBLE','SS_DOUBLE','SS_DOUBLE','SS_DOUBLE','SS_DOUBLE','SS_DOUBLE','SS_DOUBLE','SS_DOUBLE','SS_DOUBLE','SS_DOUBLE','SS_DOUBLE','SS_DOUBLE','SS_DOUBLE','SS_DOUBLE','SS_DOUBLE','SS_DOUBLE','SS_DOUBLE','SS_DOUBLE','SS_DOUBLE','SS_DOUBLE','SS_DOUBLE','SS_DOUBLE','SS_DOUBLE','SS_DOUBLE','SS_DOUBLE','SS_DOUBLE','SS_DOUBLE','SS_DOUBLE','SS_DOUBLE','SS_DOUBLE','SS_DOUBLE','SS_DOUBLE','SS_DOUBLE','SS_DOUBLE','SS_DOUBLE','SS_DOUBLE','SS_DOUBLE','SS_DOUBLE','SS_DOUBLE','SS_DOUBLE','SS_DOUBLE','SS_DOUBLE','SS_DOUBLE','SS_DOUBLE','SS_DOUBLE','SS_DOUBLE','SS_DOUBLE','SS_DOUBLE','SS_DOUBLE','SS_DOUBLE','SS_DOUBLE','SS_DOUBLE','SS_DOUBLE','SS_DOUBLE','SS_DOUBLE','SS_DOUBLE','SS_DOUBLE','SS_DOUBLE','SS_DOUBLE','SS_DOUBLE','SS_DOUBLE','SS_DOUBLE','SS_DOUBLE','SS_DOUBLE','SS_DOUBLE','SS_DOUBLE','SS_DOUBLE','SS_DOUBLE','SS_DOUBLE','SS_DOUBLE','SS_DOUBLE','SS_DOUBLE','SS_DOUBLE','SS_DOUBLE','SS_DOUBLE','SS_DOUBLE','SS_DOUBLE','SS_DOUBLE','SS_DOUBLE','SS_DOUBLE','SS_DOUBLE','SS_DOUBLE','SS_DOUBLE','SS_DOUBLE','SS_DOUBLE','SS_DOUBLE','SS_DOUBLE','SS_DOUBLE','SS_DOUBLE','SS_DOUBLE','SS_DOUBLE','SS_DOUBLE','SS_DOUBLE','SS_DOUBLE','SS_DOUBLE','SS_DOUBLE','SS_DOUBLE','SS_DOUBLE','SS_DOUBLE','SS_DOUBLE','SS_DOUBLE','SS_DOUBLE','SS_DOUBLE','SS_DOUBLE','SS_DOUBLE','SS_DOUBLE','SS_DOUBLE','SS_DOUBLE','SS_DOUBLE','SS_DOUBLE','SS_DOUBLE','SS_DOUBLE','SS_DOUBLE','SS_DOUBLE','SS_DOUBLE','SS_DOUBLE','SS_DOUBLE','SS_DOUBLE','SS_DOUBLE','SS_DOUBLE','SS_DOUBLE','SS_DOUBLE','SS_DOUBLE','SS_DOUBLE','SS_DOUBLE','SS_DOUBLE','SS_DOUBLE','SS_DOUBLE','SS_DOUBLE','SS_DOUBLE','SS_DOUBLE','SS_DOUBLE','SS_DOUBLE','SS_DOUBLE','SS_DOUBLE','SS_DOUBLE','SS_DOUBLE','SS_DOUBLE','SS_DOUBLE','SS_DOUBLE','SS_DOUBLE','SS_DOUBLE','SS_DOUBLE','SS_DOUBLE','SS_DOUBLE','SS_DOUBLE','SS_DOUBLE','SS_DOUBLE','SS_DOUBLE','SS_DOUBLE','SS_DOUBLE','SS_DOUBLE','SS_DOUBLE','SS_DOUBLE','SS_DOUBLE','SS_DOUBLE','SS_DOUBLE','SS_DOUBLE','SS_DOUBLE','SS_DOUBLE','SS_DOUBLE','SS_DOUBLE','SS_DOUBLE','SS_DOUBLE','SS_DOUBLE','SS_DOUBLE','SS_DOUBLE','SS_DOUBLE','SS_DOUBLE','SS_DOUBLE','SS_DOUBLE','SS_DOUBLE','SS_DOUBLE','SS_DOUBLE','SS_DOUBLE','SS_DOUBLE','SS_DOUBLE','SS_DOUBLE','SS_DOUBLE','SS_DOUBLE','SS_DOUBLE','SS_DOUBLE','SS_DOUBLE','SS_DOUBLE','SS_DOUBLE','SS_DOUBLE','SS_DOUBLE','SS_DOUBLE','SS_DOUBLE','SS_DOUBLE','SS_DOUBLE','SS_DOUBLE','SS_DOUBLE','SS_DOUBLE','SS_DOUBLE','SS_DOUBLE','SS_DOUBLE','SS_DOUBLE','SS_DOUBLE','SS_DOUBLE','SS_DOUBLE','SS_DOUBLE','SS_DOUBLE','SS_DOUBLE','SS_DOUBLE','SS_DOUBLE','SS_DOUBLE','SS_DOUBLE','SS_DOUBLE','SS_DOUBLE','SS_DOUBLE','SS_DOUBLE','SS_DOUBLE','SS_DOUBLE','SS_DOUBLE','SS_DOUBLE','SS_DOUBLE','SS_DOUBLE','SS_DOUBLE','SS_DOUBLE','SS_DOUBLE','SS_DOUBLE','SS_DOUBLE','SS_DOUBLE','SS_DOUBLE','SS_DOUBLE','SS_DOUBLE','SS_DOUBLE','SS_DOUBLE','SS_DOUBLE','SS_DOUBLE','SS_DOUBLE','SS_DOUBLE','SS_DOUBLE','SS_DOUBLE','SS_DOUBLE','SS_DOUBLE','SS_DOUBLE','SS_DOUBLE','SS_DOUBLE','SS_DOUBLE','SS_DOUBLE','SS_DOUBLE','SS_DOUBLE','SS_DOUBLE','SS_DOUBLE','SS_DOUBLE','SS_DOUBLE','SS_DOUBLE','SS_DOUBLE','SS_DOUBLE','SS_DOUBLE','SS_DOUBLE','SS_DOUBLE','SS_DOUBLE','SS_DOUBLE'},'DataType',{['unsigned int'],['unsigned int'],['unsigned int'],['unsigned int'],['unsigned int'],['unsigned int'],['unsigned int'],['unsigned int'],['unsigned int'],['unsigned int'],['unsigned int'],['unsigned int'],['unsigned int'],['unsigned int'],['unsigned int'],['unsigned int'],['unsigned int'],['unsigned int'],['unsigned int'],['unsigned int'],['unsigned int'],['unsigned int'],['unsigned int'],['unsigned int'],['unsigned int'],['unsigned int'],['unsigned int'],['unsigned int'],['unsigned int'],['unsigned int'],['unsigned int'],['unsigned int'],['unsigned int'],['unsigned int'],['unsigned int'],['unsigned int'],['unsigned int'],['unsigned int'],['unsigned int'],['unsigned int'],['unsigned int'],['unsigned int'],['unsigned int'],['unsigned int'],['unsigned int'],['unsigned int'],['unsigned int'],['unsigned int'],['unsigned int'],['unsigned int'],['unsigned int'],['unsigned int'],['unsigned int'],['unsigned int'],['unsigned int'],['unsigned int'],['unsigned int'],['unsigned int'],['unsigned int'],['unsigned int'],['unsigned int'],['unsigned int'],['unsigned int'],['unsigned int'],['unsigned int'],['unsigned int'],['unsigned int'],['unsigned int'],['unsigned int'],['unsigned int'],['unsigned int'],['unsigned int'],['unsigned int'],['unsigned int'],['unsigned int'],['unsigned int'],['unsigned int'],['unsigned int'],['unsigned int'],['unsigned int'],['unsigned int'],['unsigned int'],['unsigned int'],['unsigned int'],['unsigned int'],['unsigned int'],['unsigned int'],['unsigned int'],['unsigned int'],['unsigned int'],['unsigned int'],['unsigned int'],['unsigned int'],['unsigned int'],['unsigned int'],['unsigned int'],['unsigned int'],['unsigned int'],['unsigned int'],['unsigned int'],['unsigned int'],['unsigned int'],['unsigned int'],['unsigned int'],['unsigned int'],['unsigned int'],['unsigned int'],['unsigned int'],['unsigned int'],['unsigned int'],['unsigned int'],['unsigned int'],['unsigned int'],['unsigned int'],['unsigned int'],['unsigned int'],['unsigned int'],['unsigned int'],['unsigned int'],['unsigned int'],['unsigned int'],['unsigned int'],['unsigned int'],['unsigned int'],['unsigned int'],['unsigned int'],['unsigned int'],['unsigned int'],['unsigned int'],['unsigned int'],['unsigned int'],['unsigned int'],['unsigned int'],['unsigned int'],['unsigned int'],['unsigned int'],['unsigned int'],['unsigned int'],['unsigned int'],['unsigned int'],['unsigned int'],['unsigned int'],['unsigned int'],['unsigned int'],['unsigned int'],['unsigned int'],['unsigned int'],['unsigned int'],['unsigned int'],['unsigned int'],['unsigned int'],['unsigned int'],['unsigned int'],['unsigned int'],['unsigned int'],['unsigned int'],['unsigned int'],['unsigned int'],['unsigned int'],['unsigned int'],['unsigned int'],['unsigned int'],['unsigned int'],['unsigned int'],['unsigned int'],['unsigned int'],['unsigned int'],['unsigned int'],['unsigned int'],['unsigned int'],['unsigned int'],['unsigned int'],['unsigned int'],['unsigned int'],['unsigned int'],['unsigned int'],['unsigned int'],['unsigned int'],['unsigned int'],['unsigned int'],['unsigned int'],['unsigned int'],['unsigned int'],['unsigned int'],['unsigned int'],['unsigned int'],['unsigned int'],['unsigned int'],['unsigned int'],['unsigned int'],['unsigned int'],['unsigned int'],['unsigned int'],['unsigned int'],['unsigned int'],['unsigned int'],['unsigned int'],['unsigned int'],['unsigned int'],['unsigned int'],['unsigned int'],['unsigned int'],['unsigned int'],['unsigned int'],['unsigned int'],['unsigned int'],['unsigned int'],['unsigned int'],['unsigned int'],['unsigned int'],['unsigned int'],['unsigned int'],['unsigned int'],['unsigned int'],['unsigned int'],['unsigned int'],['unsigned int'],['unsigned int'],['unsigned int'],['unsigned int'],['unsigned int'],['unsigned int'],['unsigned int'],['unsigned int'],['unsigned int'],['unsigned int'],['unsigned int'],['unsigned int'],['unsigned int'],['unsigned int'],['unsigned int'],['unsigned int'],['unsigned int'],['unsigned int'],['unsigned int'],['unsigned int'],['unsigned int'],['unsigned int'],['unsigned int'],['unsigned int'],['unsigned int'],['unsigned int'],['unsigned int'],['unsigned int'],['unsigned int'],['unsigned int'],['unsigned int'],['unsigned int'],['unsigned int'],['unsigned int'],['unsigned int'],['unsigned int'],['unsigned int'],['unsigned int'],['unsigned int'],['unsigned int'],['unsigned int'],['unsigned int']},'ModeValue',{0,1,2,3,4,5,6,7,8,0,1,2,3,4,5,6,7,8,0,1,2,3,4,5,6,7,8,0,1,2,3,4,5,6,7,8,0,1,2,3,4,5,6,7,8,0,1,2,3,4,5,6,7,8,0,1,2,3,4,5,6,7,8,0,1,2,3,4,5,6,7,8,0,1,2,3,4,5,6,7,8,0,1,2,3,4,5,6,7,8,0,1,2,3,4,5,6,7,8,0,1,2,3,4,5,6,7,8,0,1,2,3,4,5,6,7,8,0,1,2,3,4,5,6,7,8,0,1,2,3,4,5,6,7,8,0,1,2,3,4,5,6,7,8,0,1,2,3,4,5,6,7,8,0,1,2,3,4,5,6,7,8,0,1,2,3,4,5,6,7,8,0,1,2,3,4,5,6,7,8,0,1,2,3,4,5,6,7,8,0,1,2,3,4,5,6,7,8,0,1,2,3,4,5,6,7,8,0,1,2,3,4,5,6,7,8,0,1,2,3,4,5,6,7,8,9,0,1,2,3,4,5,6,7,8,9,0,1,2,3,4,5,6,7,8,9,0,1,2,3,4,5,6,7,8,9,-1,-1}),'StatusSelected','no','TimeSelected','no','DeltaTimeSelected','no','BytePortSelected','no','MessageLengthSelected','no','TriggerPort',struct('Selected','no','TriggerType',0),'UserCoding',struct('Selected','no','InterfaceFile','UserDecodingFile','FcnName','UserDecodeFcn','InportSelected','no','InportWidth',1,'OutportSelected','no','OutportWidth',1),'EnablePortSelected','no','UseRXService','no','BoardType','DS1','BoardNo',2,'ControllerNo',2),'OFF',[]}},'TLCFileName',{{'rtican_rx_message','OFF',[]}})  RTISFcnParameters=struct('SFcnRTICANMessage','struct','TLCFileName','char')  RTIBlockParaDefault=struct('BoardTypeNo',4302,'BoardNo',1,'ChannelNo',1,'Parameters',struct('DataFileSupport',struct('DataFileSelectedMaster',0,'DataFileSelectedLocal',0,'DataFileName','','DataFileDate','','SelectedFile',['<no file selected>']),'Options',struct('StatusSelected',1,'TimeSelected',1,'DeltaTimeSelected',1,'BytePortSelected',0,'MessageLengthSelected',0,'TriggerPort',struct('Selected',0,'TriggerType','rising'),'UserCoding',struct('Selected',0,'InterfaceFile','UserDecodingFile','FcnName','UserDecodeFcn','InportSelected',0,'InportWidth',1,'OutportSelected',0,'OutportWidth',1),'EnablePortSelected',0,'SignalOnPortnameSelected',1,'UseRXService',0),'Message',struct('MsgOnBlocknameSelected',0,'MsgName',['RX Message'],'MsgIdFormat',0,'MsgId',100,'MsgLength',8,'NumSignals',1,'SampleTime',-1,'Signal',struct('SgnName',['RX signal'],'SgnStartBit',0,'SgnLength',8,'SgnType',0,'ModeValue',-1,'DataType',0,'SLDataType','SS_DOUBLE','ByteLayout',0,'Factor',1,'Offset',0,'Min',0,'Max',255,'SgnComment',{{}},'SgnUnit',''),'MsgIdNumFormat',0,'MsgComment',{{''}}),'Version',1.2,'general',struct('isFromLib',1)),'GroupId',struct('Group',{{'RTICAN'}},'No',1,'Behavior',{{'NAMECHANGE'}},'BlockType',{{'SINK'}},'NameChangeFlag',0),'SFcnRTICANMessage',struct('MsgType','RX','MsgName',['RX Message'],'MsgIdFormat','STD','MsgId',100,'MsgLength',8,'NumSignals',1,'SampleTime',-1,'Signal',struct('SgnName',['RX signal'],'SgnStartBit',0,'SgnLength',8,'SgnType','standard','ModeValue',-1,'DataType',['unsigned int'],'ByteLayout',['little endian'],'SLDataType','SS_DOUBLE','Factor',1,'Offset',0),'StatusSelected','yes','TimeSelected','yes','DeltaTimeSelected','yes','BytePortSelected','no','MessageLengthSelected','no','EnablePortSelected','no','UserCoding',struct('Selected','no','InterfaceFile','UserDecodingFile','FcnName','UserDecodeFcn','InportSelected','no','InportWidth',1,'OutportSelected','no','OutportWidth',1),'TriggerPort',struct('Selected','no','TriggerType','rising'),'UseRXService','no','BoardType','DS4302','BoardNo',1,'ControllerNo',1,'SFcnPortType','Scalar'),'TLCFileName','rtican_rx_message')
      settings: AttributesFormatString=Group Id: RTICAN4\n
  Out1 : Outport
  wires:
  Bus Creator/1 -> Bus Selector/1  "MotionPower"
  Bus Creator1/1 -> Out1/1  "CAN_TX_TRACK_MOVING"
  Bus Selector/1 -> Bus Creator1/1  "<CAN_TX_TRACK_MOVING01>"
  Bus Selector/2 -> Bus Creator1/2  "<CAN_TX_TRACK_MOVING02>"
  Bus Selector/3 -> Bus Creator1/3  "<CAN_TX_TRACK_MOVING03>"
  Bus Selector/4 -> Bus Creator1/4  "<CAN_TX_TRACK_MOVING04>"
  Bus Selector/5 -> Bus Creator1/5  "<CAN_TX_TRACK_MOVING05>"
  Bus Selector/6 -> Bus Creator1/6  "<CAN_TX_TRACK_MOVING06>"
  Bus Selector/7 -> Bus Creator1/7  "<CAN_TX_TRACK_MOVING07>"
  Bus Selector/8 -> Bus Creator1/8  "<CAN_TX_TRACK_MOVING08>"
  Bus Selector/9 -> Bus Creator1/9  "<CAN_TX_TRACK_MOVING09>"
  Bus Selector/10 -> Bus Creator1/10  "<CAN_TX_TRACK_MOVING10>"
  Bus Selector/11 -> Bus Creator1/11  "<CAN_TX_TRACK_MOVING11>"
  Bus Selector/12 -> Bus Creator1/12  "<CAN_TX_TRACK_MOVING12>"
  Bus Selector/13 -> Bus Creator1/13  "<CAN_TX_TRACK_MOVING13>"
  Bus Selector/14 -> Bus Creator1/14  "<CAN_TX_TRACK_MOVING14>"
  Bus Selector/15 -> Bus Creator1/15  "<CAN_TX_TRACK_MOVING15>"
  Bus Selector/16 -> Bus Creator1/16  "<CAN_TX_TRACK_MOVING16>"
  Bus Selector/17 -> Bus Creator1/17  "<CAN_TX_TRACK_MOVING17>"
  Bus Selector/18 -> Bus Creator1/18  "<CAN_TX_TRACK_MOVING18>"
  Bus Selector/19 -> Bus Creator1/19  "<CAN_TX_TRACK_MOVING19>"
  Bus Selector/20 -> Bus Creator1/20  "<CAN_TX_TRACK_MOVING20>"
  Bus Selector/21 -> Bus Creator1/21  "<CAN_TX_TRACK_MOVING21>"
  Bus Selector/22 -> Bus Creator1/22  "<CAN_TX_TRACK_MOVING22>"
  Bus Selector/23 -> Bus Creator1/23  "<CAN_TX_TRACK_MOVING23>"
  Bus Selector/24 -> Bus Creator1/24  "<CAN_TX_TRACK_MOVING24>"
  Bus Selector/25 -> Bus Creator1/25  "<CAN_TX_TRACK_MOVING25>"
  Bus Selector/26 -> Bus Creator1/26  "<CAN_TX_TRACK_MOVING26>"
  Bus Selector/27 -> Bus Creator1/27  "<CAN_TX_TRACK_MOVING27>"
  Bus Selector/28 -> Bus Creator1/28  "<CAN_TX_TRACK_MOVING28>"
  Bus Selector/29 -> Bus Creator1/29  "<CAN_TX_TRACK_MOVING29>"
  Bus Selector/30 -> Bus Creator1/30  "<CAN_TX_TRACK_MOVING30>"
  Bus Selector/31 -> Bus Creator1/31  "<CAN_TX_TRACK_MOVING31>"
  Bus Selector/32 -> Bus Creator1/32  "<CAN_TX_TRACK_MOVING32>"
  Bus Selector/33 -> Bus Creator1/33  "<CAN_TX_TRACK_MOVING33>"
  Bus Selector/34 -> Bus Creator1/34  "<CAN_TX_TRACK_MOVING34>"
  Bus Selector/35 -> Bus Creator1/35  "<CAN_TX_TRACK_MOVING35>"
  Bus Selector/36 -> Bus Creator1/36  "<CAN_TX_TRACK_MOVING36>"
  Bus Selector/37 -> Bus Creator1/37  "<CAN_TX_TRACK_MOVING37>"
  Bus Selector/38 -> Bus Creator1/38  "<CAN_TX_TRACK_MOVING38>"
  Bus Selector/39 -> Bus Creator1/39  "<CAN_TX_TRACK_MOVING39>"
  Bus Selector/40 -> Bus Creator1/40  "<CAN_TX_TRACK_MOVING40>"
  Bus Selector/41 -> Bus Creator1/41  "<CAN_TX_TRACK_MOVING41>"
  Bus Selector/42 -> Bus Creator1/42  "<CAN_TX_TRACK_MOVING42>"
  Bus Selector/43 -> Bus Creator1/43  "<CAN_TX_TRACK_MOVING43>"
  Bus Selector/44 -> Bus Creator1/44  "<CAN_TX_TRACK_MOVING44>"
  Bus Selector/45 -> Bus Creator1/45  "<CAN_TX_TRACK_MOVING45>"
  Bus Selector/46 -> Bus Creator1/46  "<CAN_TX_TRACK_MOVING46>"
  Bus Selector/47 -> Bus Creator1/47  "<CAN_TX_TRACK_MOVING47>"
  Bus Selector/48 -> Bus Creator1/48  "<CAN_TX_TRACK_MOVING48>"
  Bus Selector/49 -> Bus Creator1/49  "<CAN_TX_TRACK_MOVING49>"
  Bus Selector/50 -> Bus Creator1/50  "<CAN_TX_TRACK_MOVING50>"
  Bus Selector/51 -> Bus Creator1/51  "<CAN_TX_TRACK_MOVING51>"
  Bus Selector/52 -> Bus Creator1/52  "<CAN_TX_TRACK_MOVING52>"
  Bus Selector/53 -> Bus Creator1/53  "<CAN_TX_TRACK_MOVING53>"
  Bus Selector/54 -> Bus Creator1/54  "<CAN_TX_TRACK_MOVING54>"
  Bus Selector/55 -> Bus Creator1/55  "<CAN_TX_TRACK_MOVING55>"
  Bus Selector/56 -> Bus Creator1/56  "<CAN_TX_TRACK_MOVING56>"
  Bus Selector/57 -> Bus Creator1/57  "<CAN_TX_TRACK_MOVING57>"
  Bus Selector/58 -> Bus Creator1/58  "<CAN_TX_TRACK_MOVING58>"
  Bus Selector/59 -> Bus Creator1/59  "<CAN_TX_TRACK_MOVING59>"
  Bus Selector/60 -> Bus Creator1/60  "<CAN_TX_TRACK_MOVING60>"
  Bus Selector/61 -> Bus Creator1/61  "<CAN_TX_TRACK_MOVING61>"
  Bus Selector/62 -> Bus Creator1/62  "<CAN_TX_TRACK_MOVING62>"
  Bus Selector/63 -> Bus Creator1/63  "<CAN_TX_TRACK_MOVING63>"
  Bus Selector/64 -> Bus Creator1/64  "<CAN_TX_TRACK_MOVING64>"
  ESR_TrackMotionPower/1 -> Bus Creator/1  "CAN_TX_TRACK_POWER07"
  ESR_TrackMotionPower/2 -> Bus Creator/2  "CAN_TX_TRACK_POWER14"
  ESR_TrackMotionPower/3 -> Bus Creator/3  "CAN_TX_TRACK_POWER21"
  ESR_TrackMotionPower/4 -> Bus Creator/4  "CAN_TX_TRACK_POWER28"
  ESR_TrackMotionPower/5 -> Bus Creator/5  "CAN_TX_TRACK_POWER35"
  ESR_TrackMotionPower/6 -> Bus Creator/6  "CAN_TX_TRACK_POWER42"
  ESR_TrackMotionPower/7 -> Bus Creator/7  "CAN_TX_TRACK_POWER49"
  ESR_TrackMotionPower/8 -> Bus Creator/8  "CAN_TX_TRACK_POWER56"
  ESR_TrackMotionPower/9 -> Bus Creator/9  "CAN_TX_TRACK_POWER63"
  ESR_TrackMotionPower/10 -> Bus Creator/10  "CAN_TX_TRACK_MOVING07"
  ESR_TrackMotionPower/11 -> Bus Creator/11  "CAN_TX_TRACK_MOVING14"
  ESR_TrackMotionPower/12 -> Bus Creator/12  "CAN_TX_TRACK_MOVING21"
  ESR_TrackMotionPower/13 -> Bus Creator/13  "CAN_TX_TRACK_MOVING28"
  ESR_TrackMotionPower/14 -> Bus Creator/14  "CAN_TX_TRACK_MOVING35"
  ESR_TrackMotionPower/15 -> Bus Creator/15  "CAN_TX_TRACK_MOVING42"
  ESR_TrackMotionPower/16 -> Bus Creator/16  "CAN_TX_TRACK_MOVING49"
  ESR_TrackMotionPower/17 -> Bus Creator/17  "CAN_TX_TRACK_MOVING56"
  ESR_TrackMotionPower/18 -> Bus Creator/18  "CAN_TX_TRACK_MOVING63"
  ESR_TrackMotionPower/19 -> Bus Creator/19  "CAN_TX_TRACK_MOVABLE_SLOW07"
  ESR_TrackMotionPower/20 -> Bus Creator/20  "CAN_TX_TRACK_MOVABLE_SLOW14"
  ESR_TrackMotionPower/21 -> Bus Creator/21  "CAN_TX_TRACK_MOVABLE_SLOW21"
  ESR_TrackMotionPower/22 -> Bus Creator/22  "CAN_TX_TRACK_MOVABLE_SLOW28"
  ESR_TrackMotionPower/23 -> Bus Creator/23  "CAN_TX_TRACK_MOVABLE_SLOW35"
  ESR_TrackMotionPower/24 -> Bus Creator/24  "CAN_TX_TRACK_MOVABLE_SLOW42"
  ESR_TrackMotionPower/25 -> Bus Creator/25  "CAN_TX_TRACK_MOVABLE_SLOW49"
  ESR_TrackMotionPower/26 -> Bus Creator/26  "CAN_TX_TRACK_MOVABLE_SLOW56"
  ESR_TrackMotionPower/27 -> Bus Creator/27  "CAN_TX_TRACK_MOVABLE_SLOW63"
  ESR_TrackMotionPower/28 -> Bus Creator/28  "CAN_TX_TRACK_MOVABLE_FAST07"
  ESR_TrackMotionPower/29 -> Bus Creator/29  "CAN_TX_TRACK_MOVABLE_FAST14"
  ESR_TrackMotionPower/30 -> Bus Creator/30  "CAN_TX_TRACK_MOVABLE_FAST21"
  ESR_TrackMotionPower/31 -> Bus Creator/31  "CAN_TX_TRACK_MOVABLE_FAST28"
  ESR_TrackMotionPower/32 -> Bus Creator/32  "CAN_TX_TRACK_MOVABLE_FAST35"
  ESR_TrackMotionPower/33 -> Bus Creator/33  "CAN_TX_TRACK_MOVABLE_FAST42"
  ESR_TrackMotionPower/34 -> Bus Creator/34  "CAN_TX_TRACK_MOVABLE_FAST49"
  ESR_TrackMotionPower/35 -> Bus Creator/35  "CAN_TX_TRACK_MOVABLE_FAST56"
  ESR_TrackMotionPower/36 -> Bus Creator/36  "CAN_TX_TRACK_MOVABLE_FAST63"
  ESR_TrackMotionPower/37 -> Bus Creator/37  "CAN_TX_TRACK_POWER06"
  ESR_TrackMotionPower/38 -> Bus Creator/38  "CAN_TX_TRACK_POWER13"
  ESR_TrackMotionPower/39 -> Bus Creator/39  "CAN_TX_TRACK_POWER20"
  ESR_TrackMotionPower/40 -> Bus Creator/40  "CAN_TX_TRACK_POWER27"
  ESR_TrackMotionPower/41 -> Bus Creator/41  "CAN_TX_TRACK_POWER34"
  ESR_TrackMotionPower/42 -> Bus Creator/42  "CAN_TX_TRACK_POWER41"
  ESR_TrackMotionPower/43 -> Bus Creator/43  "CAN_TX_TRACK_POWER48"
  ESR_TrackMotionPower/44 -> Bus Creator/44  "CAN_TX_TRACK_POWER55"
  ESR_TrackMotionPower/45 -> Bus Creator/45  "CAN_TX_TRACK_POWER62"
  ESR_TrackMotionPower/46 -> Bus Creator/46  "CAN_TX_TRACK_MOVING06"
  ESR_TrackMotionPower/47 -> Bus Creator/47  "CAN_TX_TRACK_MOVING13"
  ESR_TrackMotionPower/48 -> Bus Creator/48  "CAN_TX_TRACK_MOVING20"
  ESR_TrackMotionPower/49 -> Bus Creator/49  "CAN_TX_TRACK_MOVING27"
  ESR_TrackMotionPower/50 -> Bus Creator/50  "CAN_TX_TRACK_MOVING34"
  ESR_TrackMotionPower/51 -> Bus Creator/51  "CAN_TX_TRACK_MOVING41"
  ESR_TrackMotionPower/52 -> Bus Creator/52  "CAN_TX_TRACK_MOVING48"
  ESR_TrackMotionPower/53 -> Bus Creator/53  "CAN_TX_TRACK_MOVING55"
  ESR_TrackMotionPower/54 -> Bus Creator/54  "CAN_TX_TRACK_MOVING62"
  ESR_TrackMotionPower/55 -> Bus Creator/55  "CAN_TX_TRACK_MOVABLE_SLOW06"
  ESR_TrackMotionPower/56 -> Bus Creator/56  "CAN_TX_TRACK_MOVABLE_SLOW13"
  ESR_TrackMotionPower/57 -> Bus Creator/57  "CAN_TX_TRACK_MOVABLE_SLOW20"
  ESR_TrackMotionPower/58 -> Bus Creator/58  "CAN_TX_TRACK_MOVABLE_SLOW27"
  ESR_TrackMotionPower/59 -> Bus Creator/59  "CAN_TX_TRACK_MOVABLE_SLOW34"
  ESR_TrackMotionPower/60 -> Bus Creator/60  "CAN_TX_TRACK_MOVABLE_SLOW41"
  ESR_TrackMotionPower/61 -> Bus Creator/61  "CAN_TX_TRACK_MOVABLE_SLOW48"
  ESR_TrackMotionPower/62 -> Bus Creator/62  "CAN_TX_TRACK_MOVABLE_SLOW55"
  ESR_TrackMotionPower/63 -> Bus Creator/63  "CAN_TX_TRACK_MOVABLE_SLOW62"
  ESR_TrackMotionPower/64 -> Bus Creator/64  "CAN_TX_TRACK_MOVABLE_FAST06"
  ESR_TrackMotionPower/65 -> Bus Creator/65  "CAN_TX_TRACK_MOVABLE_FAST13"
  ESR_TrackMotionPower/66 -> Bus Creator/66  "CAN_TX_TRACK_MOVABLE_FAST20"
  ESR_TrackMotionPower/67 -> Bus Creator/67  "CAN_TX_TRACK_MOVABLE_FAST27"
  ESR_TrackMotionPower/68 -> Bus Creator/68  "CAN_TX_TRACK_MOVABLE_FAST34"
  ESR_TrackMotionPower/69 -> Bus Creator/69  "CAN_TX_TRACK_MOVABLE_FAST41"
  ESR_TrackMotionPower/70 -> Bus Creator/70  "CAN_TX_TRACK_MOVABLE_FAST48"
  ESR_TrackMotionPower/71 -> Bus Creator/71  "CAN_TX_TRACK_MOVABLE_FAST55"
  ESR_TrackMotionPower/72 -> Bus Creator/72  "CAN_TX_TRACK_MOVABLE_FAST62"
  ESR_TrackMotionPower/73 -> Bus Creator/73  "CAN_TX_TRACK_POWER05"
  ESR_TrackMotionPower/74 -> Bus Creator/74  "CAN_TX_TRACK_POWER12"
  ESR_TrackMotionPower/75 -> Bus Creator/75  "CAN_TX_TRACK_POWER19"
  ESR_TrackMotionPower/76 -> Bus Creator/76  "CAN_TX_TRACK_POWER26"
  ESR_TrackMotionPower/77 -> Bus Creator/77  "CAN_TX_TRACK_POWER33"
  ESR_TrackMotionPower/78 -> Bus Creator/78  "CAN_TX_TRACK_POWER40"
  ESR_TrackMotionPower/79 -> Bus Creator/79  "CAN_TX_TRACK_POWER47"
  ESR_TrackMotionPower/80 -> Bus Creator/80  "CAN_TX_TRACK_POWER54"
  ESR_TrackMotionPower/81 -> Bus Creator/81  "CAN_TX_TRACK_POWER61"
  ESR_TrackMotionPower/82 -> Bus Creator/82  "CAN_TX_TRACK_MOVING05"
  ESR_TrackMotionPower/83 -> Bus Creator/83  "CAN_TX_TRACK_MOVING12"
  ESR_TrackMotionPower/84 -> Bus Creator/84  "CAN_TX_TRACK_MOVING19"
  ESR_TrackMotionPower/85 -> Bus Creator/85  "CAN_TX_TRACK_MOVING26"
  ESR_TrackMotionPower/86 -> Bus Creator/86  "CAN_TX_TRACK_MOVING33"
  ESR_TrackMotionPower/87 -> Bus Creator/87  "CAN_TX_TRACK_MOVING40"
  ESR_TrackMotionPower/88 -> Bus Creator/88  "CAN_TX_TRACK_MOVING47"
  ESR_TrackMotionPower/89 -> Bus Creator/89  "CAN_TX_TRACK_MOVING54"
  ESR_TrackMotionPower/90 -> Bus Creator/90  "CAN_TX_TRACK_MOVING61"
  ESR_TrackMotionPower/91 -> Bus Creator/91  "CAN_TX_TRACK_MOVABLE_SLOW05"
  ESR_TrackMotionPower/92 -> Bus Creator/92  "CAN_TX_TRACK_MOVABLE_SLOW12"
  ESR_TrackMotionPower/93 -> Bus Creator/93  "CAN_TX_TRACK_MOVABLE_SLOW19"
  ESR_TrackMotionPower/94 -> Bus Creator/94  "CAN_TX_TRACK_MOVABLE_SLOW26"
  ESR_TrackMotionPower/95 -> Bus Creator/95  "CAN_TX_TRACK_MOVABLE_SLOW33"
  ESR_TrackMotionPower/96 -> Bus Creator/96  "CAN_TX_TRACK_MOVABLE_SLOW40"
  ESR_TrackMotionPower/97 -> Bus Creator/97  "CAN_TX_TRACK_MOVABLE_SLOW47"
  ESR_TrackMotionPower/98 -> Bus Creator/98  "CAN_TX_TRACK_MOVABLE_SLOW54"
  ESR_TrackMotionPower/99 -> Bus Creator/99  "CAN_TX_TRACK_MOVABLE_SLOW61"
  ESR_TrackMotionPower/100 -> Bus Creator/100  "CAN_TX_TRACK_MOVABLE_FAST05"
  ESR_TrackMotionPower/101 -> Bus Creator/101  "CAN_TX_TRACK_MOVABLE_FAST12"
  ESR_TrackMotionPower/102 -> Bus Creator/102  "CAN_TX_TRACK_MOVABLE_FAST19"
  ESR_TrackMotionPower/103 -> Bus Creator/103  "CAN_TX_TRACK_MOVABLE_FAST26"
  ESR_TrackMotionPower/104 -> Bus Creator/104  "CAN_TX_TRACK_MOVABLE_FAST33"
  ESR_TrackMotionPower/105 -> Bus Creator/105  "CAN_TX_TRACK_MOVABLE_FAST40"
  ESR_TrackMotionPower/106 -> Bus Creator/106  "CAN_TX_TRACK_MOVABLE_FAST47"
  ESR_TrackMotionPower/107 -> Bus Creator/107  "CAN_TX_TRACK_MOVABLE_FAST54"
  ESR_TrackMotionPower/108 -> Bus Creator/108  "CAN_TX_TRACK_MOVABLE_FAST61"
  ESR_TrackMotionPower/109 -> Bus Creator/109  "CAN_TX_TRACK_POWER04"
  ESR_TrackMotionPower/110 -> Bus Creator/110  "CAN_TX_TRACK_POWER11"
  ESR_TrackMotionPower/111 -> Bus Creator/111  "CAN_TX_TRACK_POWER18"
  ESR_TrackMotionPower/112 -> Bus Creator/112  "CAN_TX_TRACK_POWER25"
  ESR_TrackMotionPower/113 -> Bus Creator/113  "CAN_TX_TRACK_POWER32"
  ESR_TrackMotionPower/114 -> Bus Creator/114  "CAN_TX_TRACK_POWER39"
  ESR_TrackMotionPower/115 -> Bus Creator/115  "CAN_TX_TRACK_POWER46"
  ESR_TrackMotionPower/116 -> Bus Creator/116  "CAN_TX_TRACK_POWER53"
  ESR_TrackMotionPower/117 -> Bus Creator/117  "CAN_TX_TRACK_POWER60"
  ESR_TrackMotionPower/118 -> Bus Creator/118  "CAN_TX_TRACK_MOVING04"
  ESR_TrackMotionPower/119 -> Bus Creator/119  "CAN_TX_TRACK_MOVING11"
  ESR_TrackMotionPower/120 -> Bus Creator/120  "CAN_TX_TRACK_MOVING18"
  ESR_TrackMotionPower/121 -> Bus Creator/121  "CAN_TX_TRACK_MOVING25"
  ESR_TrackMotionPower/122 -> Bus Creator/122  "CAN_TX_TRACK_MOVING32"
  ESR_TrackMotionPower/123 -> Bus Creator/123  "CAN_TX_TRACK_MOVING39"
  ESR_TrackMotionPower/124 -> Bus Creator/124  "CAN_TX_TRACK_MOVING46"
  ESR_TrackMotionPower/125 -> Bus Creator/125  "CAN_TX_TRACK_MOVING53"
  ESR_TrackMotionPower/126 -> Bus Creator/126  "CAN_TX_TRACK_MOVING60"
  ESR_TrackMotionPower/127 -> Bus Creator/127  "CAN_TX_TRACK_MOVABLE_SLOW04"
  ESR_TrackMotionPower/128 -> Bus Creator/128  "CAN_TX_TRACK_MOVABLE_SLOW11"
  ESR_TrackMotionPower/129 -> Bus Creator/129  "CAN_TX_TRACK_MOVABLE_SLOW18"
  ESR_TrackMotionPower/130 -> Bus Creator/130  "CAN_TX_TRACK_MOVABLE_SLOW25"
  ESR_TrackMotionPower/131 -> Bus Creator/131  "CAN_TX_TRACK_MOVABLE_SLOW32"
  ESR_TrackMotionPower/132 -> Bus Creator/132  "CAN_TX_TRACK_MOVABLE_SLOW39"
  ESR_TrackMotionPower/133 -> Bus Creator/133  "CAN_TX_TRACK_MOVABLE_SLOW46"
  ESR_TrackMotionPower/134 -> Bus Creator/134  "CAN_TX_TRACK_MOVABLE_SLOW53"
  ESR_TrackMotionPower/135 -> Bus Creator/135  "CAN_TX_TRACK_MOVABLE_SLOW60"
  ESR_TrackMotionPower/136 -> Bus Creator/136  "CAN_TX_TRACK_MOVABLE_FAST04"
  ESR_TrackMotionPower/137 -> Bus Creator/137  "CAN_TX_TRACK_MOVABLE_FAST11"
  ESR_TrackMotionPower/138 -> Bus Creator/138  "CAN_TX_TRACK_MOVABLE_FAST18"
  ESR_TrackMotionPower/139 -> Bus Creator/139  "CAN_TX_TRACK_MOVABLE_FAST25"
  ESR_TrackMotionPower/140 -> Bus Creator/140  "CAN_TX_TRACK_MOVABLE_FAST32"
  ESR_TrackMotionPower/141 -> Bus Creator/141  "CAN_TX_TRACK_MOVABLE_FAST39"
  ESR_TrackMotionPower/142 -> Bus Creator/142  "CAN_TX_TRACK_MOVABLE_FAST46"
  ESR_TrackMotionPower/143 -> Bus Creator/143  "CAN_TX_TRACK_MOVABLE_FAST53"
  ESR_TrackMotionPower/144 -> Bus Creator/144  "CAN_TX_TRACK_MOVABLE_FAST60"
  ESR_TrackMotionPower/145 -> Bus Creator/145  "CAN_TX_TRACK_POWER03"
  ESR_TrackMotionPower/146 -> Bus Creator/146  "CAN_TX_TRACK_POWER10"
  ESR_TrackMotionPower/147 -> Bus Creator/147  "CAN_TX_TRACK_POWER17"
  ESR_TrackMotionPower/148 -> Bus Creator/148  "CAN_TX_TRACK_POWER24"
  ESR_TrackMotionPower/149 -> Bus Creator/149  "CAN_TX_TRACK_POWER31"
  ESR_TrackMotionPower/150 -> Bus Creator/150  "CAN_TX_TRACK_POWER38"
  ESR_TrackMotionPower/151 -> Bus Creator/151  "CAN_TX_TRACK_POWER45"
  ESR_TrackMotionPower/152 -> Bus Creator/152  "CAN_TX_TRACK_POWER52"
  ESR_TrackMotionPower/153 -> Bus Creator/153  "CAN_TX_TRACK_POWER59"
  ESR_TrackMotionPower/154 -> Bus Creator/154  "CAN_TX_TRACK_MOVING03"
  ESR_TrackMotionPower/155 -> Bus Creator/155  "CAN_TX_TRACK_MOVING10"
  ESR_TrackMotionPower/156 -> Bus Creator/156  "CAN_TX_TRACK_MOVING17"
  ESR_TrackMotionPower/157 -> Bus Creator/157  "CAN_TX_TRACK_MOVING24"
  ESR_TrackMotionPower/158 -> Bus Creator/158  "CAN_TX_TRACK_MOVING31"
  ESR_TrackMotionPower/159 -> Bus Creator/159  "CAN_TX_TRACK_MOVING38"
  ESR_TrackMotionPower/160 -> Bus Creator/160  "CAN_TX_TRACK_MOVING45"
  ESR_TrackMotionPower/161 -> Bus Creator/161  "CAN_TX_TRACK_MOVING52"
  ESR_TrackMotionPower/162 -> Bus Creator/162  "CAN_TX_TRACK_MOVING59"
  ESR_TrackMotionPower/163 -> Bus Creator/163  "CAN_TX_TRACK_MOVABLE_SLOW03"
  ESR_TrackMotionPower/164 -> Bus Creator/164  "CAN_TX_TRACK_MOVABLE_SLOW10"
  ESR_TrackMotionPower/165 -> Bus Creator/165  "CAN_TX_TRACK_MOVABLE_SLOW17"
  ESR_TrackMotionPower/166 -> Bus Creator/166  "CAN_TX_TRACK_MOVABLE_SLOW24"
  ESR_TrackMotionPower/167 -> Bus Creator/167  "CAN_TX_TRACK_MOVABLE_SLOW31"
  ESR_TrackMotionPower/168 -> Bus Creator/168  "CAN_TX_TRACK_MOVABLE_SLOW38"
  ESR_TrackMotionPower/169 -> Bus Creator/169  "CAN_TX_TRACK_MOVABLE_SLOW45"
  ESR_TrackMotionPower/170 -> Bus Creator/170  "CAN_TX_TRACK_MOVABLE_SLOW52"
  ESR_TrackMotionPower/171 -> Bus Creator/171  "CAN_TX_TRACK_MOVABLE_SLOW59"
  ESR_TrackMotionPower/172 -> Bus Creator/172  "CAN_TX_TRACK_MOVABLE_FAST03"
  ESR_TrackMotionPower/173 -> Bus Creator/173  "CAN_TX_TRACK_MOVABLE_FAST10"
  ESR_TrackMotionPower/174 -> Bus Creator/174  "CAN_TX_TRACK_MOVABLE_FAST17"
  ESR_TrackMotionPower/175 -> Bus Creator/175  "CAN_TX_TRACK_MOVABLE_FAST24"
  ESR_TrackMotionPower/176 -> Bus Creator/176  "CAN_TX_TRACK_MOVABLE_FAST31"
  ESR_TrackMotionPower/177 -> Bus Creator/177  "CAN_TX_TRACK_MOVABLE_FAST38"
  ESR_TrackMotionPower/178 -> Bus Creator/178  "CAN_TX_TRACK_MOVABLE_FAST45"
  ESR_TrackMotionPower/179 -> Bus Creator/179  "CAN_TX_TRACK_MOVABLE_FAST52"
  ESR_TrackMotionPower/180 -> Bus Creator/180  "CAN_TX_TRACK_MOVABLE_FAST59"
  ESR_TrackMotionPower/181 -> Bus Creator/181  "CAN_TX_TRACK_POWER02"
  ESR_TrackMotionPower/182 -> Bus Creator/182  "CAN_TX_TRACK_POWER09"
  ESR_TrackMotionPower/183 -> Bus Creator/183  "CAN_TX_TRACK_POWER16"
  ESR_TrackMotionPower/184 -> Bus Creator/184  "CAN_TX_TRACK_POWER23"
  ESR_TrackMotionPower/185 -> Bus Creator/185  "CAN_TX_TRACK_POWER30"
  ESR_TrackMotionPower/186 -> Bus Creator/186  "CAN_TX_TRACK_POWER37"
  ESR_TrackMotionPower/187 -> Bus Creator/187  "CAN_TX_TRACK_POWER44"
  ESR_TrackMotionPower/188 -> Bus Creator/188  "CAN_TX_TRACK_POWER51"
  ESR_TrackMotionPower/189 -> Bus Creator/189  "CAN_TX_TRACK_POWER58"
  ESR_TrackMotionPower/190 -> Bus Creator/190  "CAN_TX_TRACK_MOVING02"
  ESR_TrackMotionPower/191 -> Bus Creator/191  "CAN_TX_TRACK_MOVING09"
  ESR_TrackMotionPower/192 -> Bus Creator/192  "CAN_TX_TRACK_MOVING16"
  ESR_TrackMotionPower/193 -> Bus Creator/193  "CAN_TX_TRACK_MOVING23"
  ESR_TrackMotionPower/194 -> Bus Creator/194  "CAN_TX_TRACK_MOVING30"
  ESR_TrackMotionPower/195 -> Bus Creator/195  "CAN_TX_TRACK_MOVING37"
  ESR_TrackMotionPower/196 -> Bus Creator/196  "CAN_TX_TRACK_MOVING44"
  ESR_TrackMotionPower/197 -> Bus Creator/197  "CAN_TX_TRACK_MOVING51"
  ESR_TrackMotionPower/198 -> Bus Creator/198  "CAN_TX_TRACK_MOVING58"
  ESR_TrackMotionPower/199 -> Bus Creator/199  "CAN_TX_TRACK_MOVABLE_SLOW02"
  ESR_TrackMotionPower/200 -> Bus Creator/200  "CAN_TX_TRACK_MOVABLE_SLOW09"
  ESR_TrackMotionPower/201 -> Bus Creator/201  "CAN_TX_TRACK_MOVABLE_SLOW16"
  ESR_TrackMotionPower/202 -> Bus Creator/202  "CAN_TX_TRACK_MOVABLE_SLOW23"
  ESR_TrackMotionPower/203 -> Bus Creator/203  "CAN_TX_TRACK_MOVABLE_SLOW30"
  ESR_TrackMotionPower/204 -> Bus Creator/204  "CAN_TX_TRACK_MOVABLE_SLOW37"
  ESR_TrackMotionPower/205 -> Bus Creator/205  "CAN_TX_TRACK_MOVABLE_SLOW44"
  ESR_TrackMotionPower/206 -> Bus Creator/206  "CAN_TX_TRACK_MOVABLE_SLOW51"
  ESR_TrackMotionPower/207 -> Bus Creator/207  "CAN_TX_TRACK_MOVABLE_SLOW58"
  ESR_TrackMotionPower/208 -> Bus Creator/208  "CAN_TX_TRACK_MOVABLE_FAST02"
  ESR_TrackMotionPower/209 -> Bus Creator/209  "CAN_TX_TRACK_MOVABLE_FAST09"
  ESR_TrackMotionPower/210 -> Bus Creator/210  "CAN_TX_TRACK_MOVABLE_FAST16"
  ESR_TrackMotionPower/211 -> Bus Creator/211  "CAN_TX_TRACK_MOVABLE_FAST23"
  ESR_TrackMotionPower/212 -> Bus Creator/212  "CAN_TX_TRACK_MOVABLE_FAST30"
  ESR_TrackMotionPower/213 -> Bus Creator/213  "CAN_TX_TRACK_MOVABLE_FAST37"
  ESR_TrackMotionPower/214 -> Bus Creator/214  "CAN_TX_TRACK_MOVABLE_FAST44"
  ESR_TrackMotionPower/215 -> Bus Creator/215  "CAN_TX_TRACK_MOVABLE_FAST51"
  ESR_TrackMotionPower/216 -> Bus Creator/216  "CAN_TX_TRACK_MOVABLE_FAST58"
  ESR_TrackMotionPower/217 -> Bus Creator/217  "CAN_TX_TRACK_POWER01"
  ESR_TrackMotionPower/218 -> Bus Creator/218  "CAN_TX_TRACK_POWER08"
  ESR_TrackMotionPower/219 -> Bus Creator/219  "CAN_TX_TRACK_POWER15"
  ESR_TrackMotionPower/220 -> Bus Creator/220  "CAN_TX_TRACK_POWER22"
  ESR_TrackMotionPower/221 -> Bus Creator/221  "CAN_TX_TRACK_POWER29"
  ESR_TrackMotionPower/222 -> Bus Creator/222  "CAN_TX_TRACK_POWER36"
  ESR_TrackMotionPower/223 -> Bus Creator/223  "CAN_TX_TRACK_POWER43"
  ESR_TrackMotionPower/224 -> Bus Creator/224  "CAN_TX_TRACK_POWER50"
  ESR_TrackMotionPower/225 -> Bus Creator/225  "CAN_TX_TRACK_POWER57"
  ESR_TrackMotionPower/226 -> Bus Creator/226  "CAN_TX_TRACK_POWER64"
  ESR_TrackMotionPower/227 -> Bus Creator/227  "CAN_TX_TRACK_MOVING01"
  ESR_TrackMotionPower/228 -> Bus Creator/228  "CAN_TX_TRACK_MOVING08"
  ESR_TrackMotionPower/229 -> Bus Creator/229  "CAN_TX_TRACK_MOVING15"
  ESR_TrackMotionPower/230 -> Bus Creator/230  "CAN_TX_TRACK_MOVING22"
  ESR_TrackMotionPower/231 -> Bus Creator/231  "CAN_TX_TRACK_MOVING29"
  ESR_TrackMotionPower/232 -> Bus Creator/232  "CAN_TX_TRACK_MOVING36"
  ESR_TrackMotionPower/233 -> Bus Creator/233  "CAN_TX_TRACK_MOVING43"
  ESR_TrackMotionPower/234 -> Bus Creator/234  "CAN_TX_TRACK_MOVING50"
  ESR_TrackMotionPower/235 -> Bus Creator/235  "CAN_TX_TRACK_MOVING57"
  ESR_TrackMotionPower/236 -> Bus Creator/236  "CAN_TX_TRACK_MOVING64"
  ESR_TrackMotionPower/237 -> Bus Creator/237  "CAN_TX_TRACK_MOVABLE_SLOW01"
  ESR_TrackMotionPower/238 -> Bus Creator/238  "CAN_TX_TRACK_MOVABLE_SLOW08"
  ESR_TrackMotionPower/239 -> Bus Creator/239  "CAN_TX_TRACK_MOVABLE_SLOW15"
  ESR_TrackMotionPower/240 -> Bus Creator/240  "CAN_TX_TRACK_MOVABLE_SLOW22"
  ESR_TrackMotionPower/241 -> Bus Creator/241  "CAN_TX_TRACK_MOVABLE_SLOW29"
  ESR_TrackMotionPower/242 -> Bus Creator/242  "CAN_TX_TRACK_MOVABLE_SLOW36"
  ESR_TrackMotionPower/243 -> Bus Creator/243  "CAN_TX_TRACK_MOVABLE_SLOW43"
  ESR_TrackMotionPower/244 -> Bus Creator/244  "CAN_TX_TRACK_MOVABLE_SLOW50"
  ESR_TrackMotionPower/245 -> Bus Creator/245  "CAN_TX_TRACK_MOVABLE_SLOW57"
  ESR_TrackMotionPower/246 -> Bus Creator/246  "CAN_TX_TRACK_MOVABLE_SLOW64"
  ESR_TrackMotionPower/247 -> Bus Creator/247  "CAN_TX_TRACK_MOVABLE_FAST01"
  ESR_TrackMotionPower/248 -> Bus Creator/248  "CAN_TX_TRACK_MOVABLE_FAST08"
  ESR_TrackMotionPower/249 -> Bus Creator/249  "CAN_TX_TRACK_MOVABLE_FAST15"
  ESR_TrackMotionPower/250 -> Bus Creator/250  "CAN_TX_TRACK_MOVABLE_FAST22"
  ESR_TrackMotionPower/251 -> Bus Creator/251  "CAN_TX_TRACK_MOVABLE_FAST29"
  ESR_TrackMotionPower/252 -> Bus Creator/252  "CAN_TX_TRACK_MOVABLE_FAST36"
  ESR_TrackMotionPower/253 -> Bus Creator/253  "CAN_TX_TRACK_MOVABLE_FAST43"
  ESR_TrackMotionPower/254 -> Bus Creator/254  "CAN_TX_TRACK_MOVABLE_FAST50"
  ESR_TrackMotionPower/255 -> Bus Creator/255  "CAN_TX_TRACK_MOVABLE_FAST57"
  ESR_TrackMotionPower/256 -> Bus Creator/256  "CAN_TX_TRACK_MOVABLE_FAST64"
  ESR_TrackMotionPower/257 -> Bus Creator/257  "CAN_TX_TRACK_CAN_ID_GROUP"
  ESR_TrackMotionPower/258 -> Bus Creator/258  "CAN_TX_TRACK_ROLLING_COUNT_2"
